simulink model "vehicle_dynamics_system"  (R2012b)
settings: Solver=ode3  StartTime=0.0  StopTime=10.0  FixedStep=T  RelTol=1e-3
PreLoadFcn:
  | init_parameters;
undefined symbols (not defined in the file): CarBody, Differential, Engine, Gearbox, Ground, Suspension, Wheel
libraries: vehicle_dynamics_lib x11, simulink x1
(part 2 of 3)

== matlab function vehicle_dynamics_system/Chassis/Vehicle dynamics ==
  data: q input size=16; q2dot output size=16; stuck output; q1dot input size=16; r_DFL input; FTireFL input; r_DFR input; FTireFR input; r_DRL input; FTireRL input; r_DRR input; FTireRR input; FDamperFL input; FDamperFR input; FDamperRL input; FDamperRR input; gravity input; rFLWheelMountPoint parameter; rFRWheelMountPoint parameter; rRLWheelMountPoint parameter; rRRWheelMountPoint parameter; delta input; rFAirPointOfAttack parameter; rRAirPointOfAttack parameter; FAirDrag input; M_FL input; M_FR input; M_RL input; M_RR input; c_ROLLBARF parameter; c_ROLLBARR parameter; M_BrakeF input; M_BrakeR input; R output; N_Gnd input; m_body parameter; m_wheel parameter; I_body parameter; I_wheel parameter
function [q2dot, stuck, R] ...
    = vehicle_dynamics(q, q1dot, r_DFL, FTireFL, r_DFR, FTireFR, r_DRL, FTireRL, ...
    r_DRR, FTireRR, FDamperFL, FDamperFR, FDamperRL, FDamperRR, gravity, rFLWheelMountPoint, ...
    rFRWheelMountPoint, rRLWheelMountPoint, rRRWheelMountPoint, delta, ...
    rFAirPointOfAttack, rRAirPointOfAttack, FAirDrag, M_FL, M_FR, M_RL, M_RR, ...
    c_ROLLBARF, c_ROLLBARR, M_BrakeF, M_BrakeR, N_Gnd, m_body, m_wheel, I_body, I_wheel)
% This block supports the Embedded MATLAB subset.
% See the help menu for details. 

persistent oldepsFL_zs1dot; if isempty(oldepsFL_zs1dot), oldepsFL_zs1dot = 0; end
persistent oldepsFR_zs1dot; if isempty(oldepsFR_zs1dot), oldepsFR_zs1dot = 0; end
persistent oldepsRL_zs1dot; if isempty(oldepsRL_zs1dot), oldepsRL_zs1dot = 0; end
persistent oldepsRR_zs1dot; if isempty(oldepsRR_zs1dot), oldepsRR_zs1dot = 0; end
persistent stuckFL; if isempty(stuckFL), stuckFL = 0; end
persistent stuckFR; if isempty(stuckFR), stuckFR = 0; end
persistent stuckRL; if isempty(stuckRL), stuckRL = 0; end
persistent stuckRR; if isempty(stuckRR), stuckRR = 0; end

% x_zs = q(1);
% y_zs = q(2);
% z_zs = q(3);
psi_zs = q(4);
theta_zs = q(5);
phi_zs = q(6);
deltaFL_zs = q(7);
deltaFR_zs = q(8);
zFL_zs = q(9);
zFR_zs = q(10);
zRL_zs = q(11);
zRR_zs = q(12);
epsFL_zs = q(13);
epsFR_zs = q(14);
epsRL_zs = q(15);
epsRR_zs = q(16);

% x_zs1dot = q1dot(1);
% y_zs1dot = q1dot(2);
% z_zs1dot = q1dot(3);
psi_zs1dot = q1dot(4);
theta_zs1dot = q1dot(5);
phi_zs1dot = q1dot(6);
deltaFL_zs1dot = q1dot(7);
deltaFR_zs1dot = q1dot(8);
zFL_zs1dot = q1dot(9);
zFR_zs1dot = q1dot(10);
zRL_zs1dot = q1dot(11);
zRR_zs1dot = q1dot(12);
epsFL_zs1dot = q1dot(13);
epsFR_zs1dot = q1dot(14);
epsRL_zs1dot = q1dot(15);
epsRR_zs1dot = q1dot(16);

xTireFL = FTireFL(1);
yTireFL = FTireFL(2);
zTireFL = FTireFL(3);

xTireFR = FTireFR(1);
yTireFR = FTireFR(2);
zTireFR = FTireFR(3);

xTireRL = FTireRL(1);
yTireRL = FTireRL(2);
zTireRL = FTireRL(3);

xTireRR = FTireRR(1);
yTireRR = FTireRR(2);
zTireRR = FTireRR(3);

%Calculate anti roll bar forces
dsuspF = zFL_zs - zFR_zs;
dsuspR = zRL_zs - zRR_zs;

F_RBF = dsuspF*c_ROLLBARF;
F_RBR = dsuspR*c_ROLLBARR;

%Calculate chassis rotation matrix
R=zeros(3,3);

t1 = cos(psi_zs);
t2 = cos(theta_zs);
t4 = sin(psi_zs);
t5 = cos(phi_zs);
t7 = sin(theta_zs);
t8 = t1 * t7;
t9 = sin(phi_zs);
t17 = t7 * t4;
R(1,1) = t1 * t2;
R(1,2) = -t4 * t5 + t8 * t9;
R(1,3) = t4 * t9 + t8 * t5;
R(2,1) = t2 * t4;
R(2,2) = t1 * t5 + t17 * t9;
R(2,3) = -t1 * t9 + t17 * t5;
R(3,1) = -t7;
R(3,2) = t2 * t9;
R(3,3) = t2 * t5;

cd = cos(deltaFL_zs);
sd = sin(deltaFL_zs);
%Calculate front wheel rotation matrix
Rf = R*[cd, -sd, 0;
        sd, cd, 0;
        0, 0, 1];

%Calculate necessary braking torque
r_fwdF = Rf(:,1);
r_fwdR = R(:,1);

if( M_BrakeF > 0 || M_BrakeR > 0 )
    
    whltrqFL = -FTireFL.'*r_fwdF*r_DFL+M_FL;
	whltrqFR = -FTireFR.'*r_fwdF*r_DFR+M_FR;
	whltrqRL = -FTireRL.'*r_fwdR*r_DRL+M_RL;
	whltrqRR = -FTireRR.'*r_fwdR*r_DRR+M_RR;
    
	M_FL = M_FL - sign(epsFL_zs1dot)*M_BrakeF;
    M_FR = M_FR - sign(epsFR_zs1dot)*M_BrakeF;
    M_RL = M_RL - sign(epsRL_zs1dot)*M_BrakeR;
    M_RR = M_RR - sign(epsRR_zs1dot)*M_BrakeR;
    
    %FL
    if( abs(whltrqFL) < M_BrakeF )
        if( sign(oldepsFL_zs1dot) ~= sign(epsFL_zs1dot) )
            stuckFL = 1;
        end
    else
        stuckFL = 0;
    end
    
    %FR
    if( abs(whltrqFR) < M_BrakeF )
        if( sign(oldepsFR_zs1dot) ~= sign(epsFR_zs1dot) )
            stuckFR = 1;
        end
    else
        stuckFR = 0;
    end
    
    %RL
    if( abs(whltrqRL) < M_BrakeR )
        if( sign(oldepsRL_zs1dot) ~= sign(epsRL_zs1dot) )
            stuckRL = 1;
        end
    else
        stuckRL = 0;
    end
    
    %RR
    if( abs(whltrqRR) < M_BrakeR )
        if( sign(oldepsRR_zs1dot) ~= sign(epsRR_zs1dot) )
            stuckRR = 1;
        end
    else
        stuckRR = 0;
    end
else
    stuckFL = 0;
    stuckFR = 0;
    stuckRL = 0;
    stuckRR = 0;
end
    
g = gravity;

n_gndFL_X = N_Gnd(1);
n_gndFL_Y = N_Gnd(2);
n_gndFL_Z = N_Gnd(3);

n_gndFR_X = N_Gnd(4);
n_gndFR_Y = N_Gnd(5);
n_gndFR_Z = N_Gnd(6);

n_gndRL_X = N_Gnd(7);
n_gndRL_Y = N_Gnd(8);
n_gndRL_Z = N_Gnd(9);

n_gndRR_X = N_Gnd(10);
n_gndRR_Y = N_Gnd(11);
n_gndRR_Z = N_Gnd(12);

F_DSFL = FDamperFL + F_RBF;
F_DSFR = FDamperFR - F_RBF;
F_DSRL = FDamperRL + F_RBR;
F_DSRR = FDamperRR - F_RBF;

F_AIRFRONT_X = FAirDrag(1);
F_AIRFRONT_Z = FAirDrag(2);

F_AIRREAR_X = FAirDrag(3);
F_AIRREAR_Z = FAirDrag(4);

r_wheelMntFL_X = rFLWheelMountPoint(1);
r_wheelMntFL_Y = rFLWheelMountPoint(2);
r_wheelMntFL_Z = rFLWheelMountPoint(3);

r_wheelMntFR_X = rFRWheelMountPoint(1);
r_wheelMntFR_Y = rFRWheelMountPoint(2);
r_wheelMntFR_Z = rFRWheelMountPoint(3);

r_wheelMntRL_X = rRLWheelMountPoint(1);
r_wheelMntRL_Y = rRLWheelMountPoint(2);
r_wheelMntRL_Z = rRLWheelMountPoint(3);

r_wheelMntRR_X = rRRWheelMountPoint(1);
r_wheelMntRR_Y = rRRWheelMountPoint(2);
r_wheelMntRR_Z = rRRWheelMountPoint(3);

r_airFront_X = rFAirPointOfAttack(1);
r_airFront_Y = rFAirPointOfAttack(2);
r_airFront_Z = rFAirPointOfAttack(3);

r_airRear_X = rRAirPointOfAttack(1);
r_airRear_Y = rRAirPointOfAttack(2);
r_airRear_Z = rRAirPointOfAttack(3);

I_body_xx = I_body(1,1);
I_body_yy = I_body(2,2);
I_body_zz = I_body(3,3);

I_wheel_xx = I_wheel(1,1);
I_wheel_yy = I_wheel(2,2);
I_wheel_zz = I_wheel(3,3);

deltaFR = delta;
deltaFL = delta;

gg = zeros(14,15);

%Warning: the function names {F_AIRFRONT_Z, F_AIRREAR_Z, M_FL, F_DSFR, F_DSRL, F_DSRR, F_AIRFRONT_X, M_FR, F_DSFL, F_AIRREAR_X, xTireFL, yTireFL, zTireFL, M_RL, M_RR, xTireFR, yTireFR, zTireFR, xTireRL, yTireRL, zTireRL, xTireRR, yTireRR, zTireRR} are not recognized in the target language
t2 = m_body + 4 * m_wheel;
t3 = m_wheel * r_wheelMntRL_Z;
t4 = sin(psi_zs);
t5 = sin(theta_zs);
t6 = t4 * t5;
t7 = cos(phi_zs);
t8 = t6 * t7;
t10 = m_wheel * zRL_zs;
t12 = cos(psi_zs);
t13 = sin(phi_zs);
t14 = t12 * t13;
t16 = m_wheel * zFR_zs;
t18 = m_wheel * r_wheelMntFL_Y;
t19 = t12 * t7;
t21 = m_wheel * t4;
t22 = cos(theta_zs);
t23 = t22 * r_wheelMntRR_X;
t25 = m_wheel * r_wheelMntRR_Y;
t27 = t22 * r_wheelMntFL_X;
t29 = m_wheel * zFL_zs;
t31 = m_wheel * r_wheelMntFR_Y;
t32 = t6 * t13;
t34 = m_wheel * r_wheelMntFR_Z;
t36 = t22 * r_wheelMntFR_X;
t39 = m_wheel * zRR_zs;
t41 = -t3 * t8 - t10 * t8 + t3 * t14 + t16 * t14 - t18 * t19 - t21 * t23 - t25 * t19 - t21 * t27 + t29 * t14 - t31 * t32 + t34 * t14 - t21 * t36 - t31 * t19 + t39 * t14;
t43 = t22 * r_wheelMntRL_X;
t45 = m_wheel * r_wheelMntRL_Y;
t49 = m_wheel * r_wheelMntFL_Z;
t51 = m_wheel * r_wheelMntRR_Z;
t60 = t10 * t14 - t21 * t43 - t45 * t19 - t16 * t8 - t34 * t8 - t49 * t8 + t51 * t14 - t18 * t32 - t45 * t32 - t29 * t8 + t49 * t14 - t51 * t8 - t25 * t32 - t39 * t8;
t61 = t41 + t60;
t62 = t12 * t22;
t63 = t62 * t7;
t65 = t62 * t13;
t68 = m_wheel * t12;
t69 = t5 * r_wheelMntFR_X;
t76 = t5 * r_wheelMntRL_X;
t80 = t5 * r_wheelMntFL_X;
t83 = t5 * r_wheelMntRR_X;
t86 = t16 * t63 + t25 * t65 + t34 * t63 - t68 * t69 + t31 * t65 + t39 * t63 + t3 * t63 + t10 * t63 + t45 * t65 - t68 * t76 + t29 * t63 + t18 * t65 - t68 * t80 + t49 * t63 - t68 * t83 + t51 * t63;
t87 = t4 * t7;
t90 = t4 * t13;
t92 = t12 * t5;
t93 = t92 * t13;
t96 = t92 * t7;
t104 = t29 * t87 + t49 * t87 + t31 * t90 - t16 * t93 - t34 * t93 + t25 * t96 + t16 * t87 + t31 * t96 - t39 * t93 + t39 * t87 + t45 * t96 - t3 * t93;
t117 = -t10 * t93 + t3 * t87 + t10 * t87 + t18 * t96 + t45 * t90 + t34 * t87 - t29 * t93 + t18 * t90 - t49 * t93 + t25 * t90 + t51 * t87 - t51 * t93;
t118 = t104 + t117;
t119 = t5 * t7;
t122 = t68 * t119 + t21 * t13;
t123 = m_wheel * zFR_zs1dot;
t124 = t87 * phi_zs1dot;
t127 = t31 * t12;
t128 = psi_zs1dot ^ 2;
t129 = t128 * t5;
t130 = t129 * t13;
t132 = t31 * t4;
t133 = psi_zs1dot * t22;
t134 = theta_zs1dot * t13;
t135 = t133 * t134;
t138 = t25 * t12;
t139 = psi_zs1dot * t13;
t140 = t139 * phi_zs1dot;
t143 = t4 * t128;
t144 = t143 * t7;
t146 = t143 * t13;
t148 = phi_zs1dot ^ 2;
t149 = t90 * t148;
t151 = t39 * t12;
t152 = psi_zs1dot * t7;
t153 = t152 * phi_zs1dot;
t156 = t18 * t12;
t159 = m_wheel * zFL_zs1dot;
t161 = t12 * psi_zs1dot * t13;
t164 = theta_zs1dot ^ 2;
t165 = t22 * t164;
t166 = t165 * r_wheelMntRR_X;
t168 = t49 * t4;
t169 = theta_zs1dot * t7;
t170 = t133 * t169;
t173 = psi_zs1dot * t5;
t174 = t13 * phi_zs1dot;
t175 = t173 * t174;
t178 = t49 * t12;
t181 = t5 * t13;
t182 = t181 * t148;
t184 = t25 * t4;
t187 = t7 * phi_zs1dot;
t188 = t173 * t187;
t191 = t128 * t22;
t192 = t191 * r_wheelMntFL_X;
t194 = 0.2e1 * t123 * t124 - t127 * t130 - 0.2e1 * t132 * t135 + 0.2e1 * t138 * t140 + t31 * t144 - t39 * t146 - t39 * t149 + 0.2e1 * t151 * t153 + 0.2e1 * t156 * t140 + 0.2e1 * t159 * t161 - t68 * t166 - 0.2e1 * t168 * t170 + 0.2e1 * t168 * t175 + 0.2e1 * t178 * t153 - t156 * t182 - 0.2e1 * t184 * t135 - 0.2e1 * t184 * t188 - t68 * t192;
t198 = t34 * t12;
t199 = t119 * t148;
t202 = t191 * r_wheelMntFR_X;
t204 = t45 * t12;
t206 = t45 * t4;
t211 = m_wheel * zRL_zs1dot;
t212 = t211 * t12;
t213 = t181 * phi_zs1dot;
t218 = t16 * t12;
t219 = t129 * t7;
t221 = t165 * r_wheelMntFR_X;
t225 = t5 * t164;
t226 = t225 * t13;
t228 = t22 * theta_zs1dot;
t229 = t228 * t187;
t232 = t225 * t7;
t237 = 0.2e1 * t127 * t140 - t34 * t146 - t198 * t199 - t16 * t146 - t68 * t202 - t204 * t130 - 0.2e1 * t206 * t135 - 0.2e1 * t206 * t188 - 0.2e1 * t212 * t213 - t49 * t149 - t49 * t146 - t218 * t219 - t68 * t221 - 0.2e1 * t132 * t188 - t127 * t226 + 0.2e1 * t127 * t229 - t151 * t232 - t127 * t182 + 0.2e1 * t198 * t153;
t240 = t29 * t4;
t246 = xTireFL;
t247 = t34 * t4;
t253 = t18 * t4;
t261 = m_wheel * zRR_zs1dot;
t262 = t261 * t4;
t263 = t173 * t7;
t266 = t261 * t12;
t267 = t228 * t7;
t272 = t51 * t12;
t273 = t228 * t174;
t282 = -t198 * t219 - 0.2e1 * t240 * t170 + 0.2e1 * t240 * t175 - t204 * t226 - t246 - 0.2e1 * t247 * t170 + 0.2e1 * t247 * t175 - t178 * t199 - 0.2e1 * t253 * t135 - 0.2e1 * t253 * t188 - t156 * t226 + 0.2e1 * t218 * t153 - 0.2e1 * t262 * t263 + 0.2e1 * t266 * t267 - 0.2e1 * t266 * t213 - 0.2e1 * t272 * t273 - 0.2e1 * t151 * t273 + 0.2e1 * t156 * t229 + 0.2e1 * t211 * t161;
t285 = t191 * r_wheelMntRL_X;
t288 = t10 * t12;
t292 = t21 * psi_zs1dot;
t293 = t5 * theta_zs1dot;
t294 = t293 * r_wheelMntRL_X;
t297 = t3 * t12;
t299 = t87 * t148;
t302 = t123 * t4;
t305 = t123 * t12;
t312 = t16 * t4;
t316 = t3 * t4;
t321 = t29 * t12;
t323 = 0.2e1 * t211 * t124 - t68 * t285 - t138 * t130 - 0.2e1 * t288 * t273 - t288 * t199 + 0.2e1 * t292 * t294 - t297 * t219 + t18 * t299 - t178 * t219 - 0.2e1 * t302 * t263 + 0.2e1 * t305 * t267 - 0.2e1 * t305 * t213 + t31 * t299 - t151 * t219 - 0.2e1 * t312 * t170 - t272 * t199 - 0.2e1 * t316 * t170 + 0.2e1 * t316 * t175 - t321 * t199;
t329 = t293 * r_wheelMntFL_X;
t332 = t39 * t4;
t338 = t51 * t4;
t341 = F_AIRFRONT_Z;
t342 = t341 * t12;
t345 = t10 * t4;
t351 = t191 * r_wheelMntRR_X;
t360 = -t178 * t232 - 0.2e1 * t178 * t273 + 0.2e1 * t292 * t329 - 0.2e1 * t332 * t170 + 0.2e1 * t332 * t175 - t272 * t219 - 0.2e1 * t338 * t170 - t342 * t119 - t288 * t219 - 0.2e1 * t345 * t170 + 0.2e1 * t345 * t175 + t25 * t144 - t68 * t351 + t25 * t299 - t51 * t146 + 0.2e1 * t338 * t175 + 0.2e1 * t261 * t124 + t45 * t144;
t361 = t165 * r_wheelMntRL_X;
t379 = t293 * r_wheelMntFR_X;
t387 = xTireRL;
t388 = xTireFR;
t389 = F_AIRREAR_Z;
t390 = t389 * t4;
t392 = -t68 * t361 - t3 * t146 - t321 * t232 - 0.2e1 * t321 * t273 + 0.2e1 * t321 * t153 + 0.2e1 * t159 * t124 - t51 * t149 + 0.2e1 * t261 * t161 - t272 * t232 - t297 * t232 - 0.2e1 * t297 * t273 - t218 * t199 + 0.2e1 * t292 * t379 + 0.2e1 * t204 * t229 - t204 * t182 + 0.2e1 * t297 * t153 - t387 - t388 - t390 * t13;
t394 = F_AIRREAR_X;
t401 = t159 * t4;
t404 = t159 * t12;
t414 = t165 * r_wheelMntFL_X;
t425 = t389 * t12;
t427 = -t62 * t394 + 0.2e1 * t204 * t140 + 0.2e1 * t288 * t153 - t3 * t149 - 0.2e1 * t401 * t263 + 0.2e1 * t404 * t267 - 0.2e1 * t404 * t213 - t321 * t219 - t29 * t149 - t198 * t232 - 0.2e1 * t198 * t273 - t68 * t414 + t18 * t144 + 0.2e1 * t312 * t175 - t218 * t232 - 0.2e1 * t218 * t273 - t34 * t149 + 0.2e1 * t123 * t161 - t425 * t119;
t439 = t211 * t4;
t445 = t293 * r_wheelMntRR_X;
t450 = xTireRR;
t452 = t341 * t4;
t454 = F_AIRFRONT_X;
t456 = -t138 * t226 - t297 * t199 - t288 * t232 - t156 * t130 - t29 * t146 - t10 * t146 - t10 * t149 + 0.2e1 * t272 * t153 - t16 * t149 + t45 * t299 - 0.2e1 * t439 * t263 + 0.2e1 * t212 * t267 - t151 * t199 + 0.2e1 * t292 * t445 + 0.2e1 * t138 * t229 - t450 - t138 * t182 - t452 * t13 - t62 * t454;
t474 = t16 * t96 + t31 * t93 + t25 * t93 + t51 * t96 + t18 * t93 + t49 * t96 + t29 * t96 + t10 * t96 + t45 * t93 + t3 * t96 + t34 * t96 - t45 * t87 + t68 * t27 - t18 * t87;
t489 = t68 * t36 - t31 * t87 + t34 * t90 + t16 * t90 + t68 * t23 - t25 * t87 + t51 * t90 + t39 * t90 + t29 * t90 + t68 * t43 + t10 * t90 + t3 * t90 + t39 * t96 + t49 * t90;
t490 = t474 + t489;
t493 = t4 * t22;
t494 = t493 * t7;
t496 = t493 * t13;
t510 = -t21 * t80 - t21 * t69 + t16 * t494 + t25 * t496 - t21 * t83 - t21 * t76 + t18 * t496 + t49 * t494 + t3 * t494 + t10 * t494 + t45 * t496 + t31 * t496 + t34 * t494 + t39 * t494 + t51 * t494 + t29 * t494;
t523 = -t29 * t19 - t18 * t14 - t31 * t14 - t34 * t19 - t16 * t19 - t34 * t32 - t16 * t32 + t25 * t8 - t25 * t14 - t51 * t19 - t39 * t19 + t18 * t8;
t536 = -t49 * t32 - t3 * t32 + t45 * t8 - t3 * t19 - t10 * t19 + t31 * t8 - t45 * t14 - t51 * t32 - t39 * t32 - t29 * t32 - t49 * t19 - t10 * t32;
t537 = t523 + t536;
t540 = t21 * t119 - t68 * t13;
t547 = t14 * t148;
t549 = t12 * t128;
t550 = t549 * t13;
t565 = yTireFL;
t567 = -0.2e1 * t272 * t175 - t338 * t232 - 0.2e1 * t338 * t273 - t338 * t199 + t10 * t547 + t10 * t550 - t316 * t219 + 0.2e1 * t266 * t263 + 0.2e1 * t262 * t267 - t206 * t226 - t206 * t130 + 0.2e1 * t204 * t135 + t51 * t550 + t51 * t547 + t39 * t547 - t184 * t130 - t565 - t132 * t130;
t576 = t68 * psi_zs1dot;
t581 = t549 * t7;
t583 = t19 * t148;
t598 = t34 * t550 + t34 * t547 + 0.2e1 * t312 * t153 - t168 * t232 - 0.2e1 * t168 * t273 - t21 * t221 - 0.2e1 * t576 * t329 - 0.2e1 * t321 * t175 - t18 * t581 - t18 * t583 + t49 * t550 - t184 * t182 - t21 * t166 - t25 * t581 + 0.2e1 * t198 * t170 - 0.2e1 * t198 * t175 - t247 * t232 - 0.2e1 * t247 * t273 + 0.2e1 * t439 * t267;
t609 = t4 * psi_zs1dot * t13;
t612 = t19 * phi_zs1dot;
t637 = -0.2e1 * t439 * t213 - t316 * t232 - 0.2e1 * t262 * t213 - t332 * t219 - 0.2e1 * t178 * t175 + 0.2e1 * t159 * t609 - 0.2e1 * t159 * t612 + 0.2e1 * t151 * t170 - 0.2e1 * t151 * t175 - 0.2e1 * t302 * t213 - t312 * t219 + 0.2e1 * t218 * t170 - 0.2e1 * t218 * t175 + 0.2e1 * t316 * t153 + 0.2e1 * t261 * t609 + t3 * t550 + 0.2e1 * t138 * t135 + 0.2e1 * t138 * t188 + 0.2e1 * t184 * t229;
t644 = yTireRR;
t664 = -t184 * t226 - 0.2e1 * t401 * t213 - t240 * t219 - t31 * t581 - t31 * t583 - t644 + 0.2e1 * t297 * t170 - 0.2e1 * t261 * t612 + t39 * t550 - t345 * t199 + t49 * t547 - t253 * t130 - t132 * t226 - t132 * t182 + 0.2e1 * t247 * t153 - t247 * t219 + 0.2e1 * t272 * t170 + 0.2e1 * t211 * t609 + 0.2e1 * t253 * t140;
t669 = yTireRL;
t697 = 0.2e1 * t404 * t263 - t669 + 0.2e1 * t401 * t267 + 0.2e1 * t156 * t135 - t312 * t232 - t312 * t199 - 0.2e1 * t576 * t379 - 0.2e1 * t211 * t612 - 0.2e1 * t332 * t273 - t332 * t232 - t332 * t199 - 0.2e1 * t576 * t445 + 0.2e1 * t184 * t140 + 0.2e1 * t332 * t153 - t390 * t119 + 0.2e1 * t204 * t188 + 0.2e1 * t127 * t135 + 0.2e1 * t127 * t188;
t723 = -t452 * t119 - 0.2e1 * t288 * t175 - t345 * t232 - 0.2e1 * t345 * t273 + t29 * t550 + t29 * t547 - t21 * t192 - t21 * t285 - t253 * t226 + 0.2e1 * t253 * t229 - t253 * t182 + 0.2e1 * t321 * t170 - t240 * t232 - t21 * t414 - t21 * t361 - t45 * t581 - t21 * t351 + 0.2e1 * t338 * t153 + 0.2e1 * t240 * t153;
t741 = yTireFR;
t754 = t16 * t550 + 0.2e1 * t123 * t609 - 0.2e1 * t123 * t612 - t21 * t202 - t316 * t199 - t345 * t219 + 0.2e1 * t288 * t170 - t493 * t454 + t425 * t13 + 0.2e1 * t212 * t263 - 0.2e1 * t316 * t273 - t741 + 0.2e1 * t178 * t170 - t45 * t583 - 0.2e1 * t576 * t294 + 0.2e1 * t206 * t140 + 0.2e1 * t132 * t140 - t247 * t199 - 0.2e1 * t312 * t273;
t783 = -t25 * t583 + 0.2e1 * t156 * t188 - t168 * t199 - 0.2e1 * t240 * t273 - t240 * t199 + 0.2e1 * t132 * t229 + 0.2e1 * t345 * t153 - 0.2e1 * t297 * t175 - t338 * t219 + 0.2e1 * t206 * t229 - t206 * t182 + t3 * t547 + 0.2e1 * t168 * t153 - t168 * t219 + t16 * t547 + 0.2e1 * t305 * t263 + 0.2e1 * t302 * t267 - t493 * t394 + t342 * t13;
t787 = m_wheel * t5;
t788 = t7 * r_wheelMntFL_Z;
t790 = t7 * zFL_zs;
t792 = m_wheel * t22;
t794 = t792 * r_wheelMntFL_X;
t795 = t7 * r_wheelMntRL_Z;
t797 = t13 * r_wheelMntFR_Y;
t799 = t7 * r_wheelMntFR_Z;
t801 = t7 * r_wheelMntRR_Z;
t803 = t7 * zRR_zs;
t805 = t7 * zFR_zs;
t807 = t13 * r_wheelMntRR_Y;
t809 = t7 * zRL_zs;
t811 = t13 * r_wheelMntRL_Y;
t813 = t13 * r_wheelMntFL_Y;
t815 = t792 * r_wheelMntRL_X;
t816 = t792 * r_wheelMntFR_X;
t817 = -t787 * t788 - t787 * t790 - t792 * r_wheelMntRR_X - t794 - t787 * t795 - t787 * t797 - t787 * t799 - t787 * t801 - t787 * t803 - t787 * t805 - t787 * t807 - t787 * t809 - t787 * t811 - t787 * t813 - t815 - t816;
t818 = t13 * r_wheelMntFL_Z;
t820 = t13 * zRR_zs;
t822 = t13 * r_wheelMntRL_Z;
t824 = t13 * zFR_zs;
t826 = t7 * r_wheelMntFR_Y;
t828 = t13 * r_wheelMntRR_Z;
t830 = t13 * r_wheelMntFR_Z;
t832 = t7 * r_wheelMntRR_Y;
t834 = t13 * zRL_zs;
t836 = t7 * r_wheelMntRL_Y;
t838 = t13 * zFL_zs;
t840 = t7 * r_wheelMntFL_Y;
t842 = -t792 * t818 - t792 * t820 - t792 * t822 - t792 * t824 + t792 * t826 - t792 * t828 - t792 * t830 + t792 * t832 - t792 * t834 + t792 * t836 - t792 * t838 + t792 * t840;
t843 = t792 * t7;
t847 = t164 * t13;
t850 = t787 * theta_zs1dot;
t854 = t164 * t7;
t867 = t7 * t148;
t870 = zTireFL;
t871 = t13 * t148;
t881 = -0.2e1 * t787 * t169 * zFL_zs1dot - t792 * t847 * r_wheelMntFL_Y - 0.2e1 * t850 * t187 * r_wheelMntFL_Y - t792 * t854 * r_wheelMntFL_Z - t792 * t847 * r_wheelMntRR_Y - 0.2e1 * t850 * t187 * r_wheelMntRR_Y - t792 * t854 * r_wheelMntRR_Z + 0.2e1 * t850 * t174 * r_wheelMntRL_Z - t792 * t867 * zFR_zs - t870 - t792 * t871 * r_wheelMntRL_Y - t792 * t854 * zRL_zs + 0.2e1 * t850 * t174 * zRL_zs - t792 * t867 * zRL_zs;
t905 = m_wheel * g;
t915 = -0.2e1 * t850 * t187 * r_wheelMntRL_Y - t792 * t854 * r_wheelMntRL_Z - 0.2e1 * t792 * t174 * zFR_zs1dot - t792 * t871 * r_wheelMntFR_Y - t792 * t847 * r_wheelMntRL_Y - 0.2e1 * t787 * t169 * zFR_zs1dot + t5 * t454 - t792 * t854 * zFR_zs - t792 * t871 * r_wheelMntRR_Y - 0.2e1 * t787 * t169 * zRR_zs1dot + (4 * t905) + 0.2e1 * t850 * t174 * r_wheelMntFL_Z - t792 * t867 * r_wheelMntFL_Z - t792 * t867 * zRR_zs + t5 * t394;
t918 = t22 * t7;
t929 = zTireFR;
t946 = (m_body * g) - t918 * t389 - t792 * t854 * r_wheelMntFR_Z + 0.2e1 * t850 * t174 * r_wheelMntFR_Z - t792 * t867 * r_wheelMntFR_Z - t792 * t854 * zFL_zs - t929 + 0.2e1 * t850 * t174 * zFL_zs - 0.2e1 * t792 * t174 * zFL_zs1dot + t787 * t164 * r_wheelMntFL_X + t787 * t164 * r_wheelMntRR_X + t787 * t164 * r_wheelMntRL_X + t787 * t164 * r_wheelMntFR_X - t792 * t867 * zFL_zs;
t964 = zTireRR;
t965 = zTireRL;
t981 = 0.2e1 * t850 * t174 * r_wheelMntRR_Z - t792 * t867 * r_wheelMntRR_Z - t792 * t854 * zRR_zs + 0.2e1 * t850 * t174 * zFR_zs - t792 * t847 * r_wheelMntFR_Y - 0.2e1 * t850 * t187 * r_wheelMntFR_Y - t792 * t871 * r_wheelMntFL_Y - t964 - t965 + 0.2e1 * t850 * t174 * zRR_zs - 0.2e1 * t792 * t174 * zRR_zs1dot - t792 * t867 * r_wheelMntRL_Z - 0.2e1 * t787 * t169 * zRL_zs1dot - 0.2e1 * t792 * t174 * zRL_zs1dot - t918 * t341;
t984 = cos(epsFL_zs);
t985 = I_wheel_zz * t984;
t986 = t985 * t22;
t987 = cos(deltaFL);
t988 = sin(epsFL_zs);
t989 = t987 * t988;
t990 = t989 * t119;
t993 = t22 ^ 2;
t994 = I_wheel_xx * t993;
t995 = cos(deltaFR);
t996 = t995 ^ 2;
t997 = cos(epsFR_zs);
t998 = t997 ^ 2;
t999 = t996 * t998;
t1002 = t987 ^ 2;
t1003 = I_wheel_zz * t1002;
t1004 = t7 ^ 2;
t1005 = t993 * t1004;
t1007 = zFL_zs ^ 2;
t1008 = m_wheel * t1007;
t1010 = r_wheelMntFL_Z ^ 2;
t1011 = m_wheel * t1010;
t1013 = t984 ^ 2;
t1014 = I_wheel_zz * t1013;
t1015 = t1002 * t993;
t1018 = I_wheel_xx * t998;
t1021 = r_wheelMntRR_Y ^ 2;
t1022 = m_wheel * t1021;
t1024 = I_wheel_zz * t1004;
t1025 = t998 * t993;
t1028 = I_wheel_xx * t1004;
t1029 = cos(epsRR_zs);
t1030 = t1029 ^ 2;
t1031 = t993 * t1030;
t1033 = r_wheelMntRL_Y ^ 2;
t1034 = m_wheel * t1033;
t1036 = I_wheel_xx * t997;
t1037 = sin(deltaFR);
t1038 = t1036 * t1037;
t1039 = sin(epsFR_zs);
t1040 = t13 * t1039;
t1041 = t7 * t993;
t1042 = t1040 * t1041;
t1045 = cos(epsRL_zs);
t1046 = t1045 ^ 2;
t1047 = I_wheel_xx * t1046;
t1048 = zRL_zs ^ 2;
t1049 = m_wheel * t1048;
t1050 = r_wheelMntFR_Y ^ 2;
t1051 = m_wheel * t1050;
t1052 = -0.2e1 * t986 * t990 - 0.2e1 * t994 * t999 + t1003 * t1005 - t1008 * t1005 - t1011 * t1005 + 0.2e1 * t1014 * t1015 - 0.2e1 * t1018 * t1005 + t1022 * t1005 + 0.2e1 * t1024 * t1025 - t1028 * t1031 + t1034 * t1005 + 0.2e1 * t1038 * t1042 + t1047 + t1049 + t1051 + t1022;
t1053 = I_wheel_yy * t1002;
t1054 = I_wheel_zz * t1030;
t1055 = I_wheel_xx * t1030;
t1056 = r_wheelMntRR_Z ^ 2;
t1057 = m_wheel * t1056;
t1058 = r_wheelMntFL_Y ^ 2;
t1059 = m_wheel * t1058;
t1060 = I_wheel_zz * t996;
t1063 = 2 * t49 * zFL_zs;
t1064 = I_wheel_zz * t993;
t1067 = t49 * t13;
t1071 = t996 * t993;
t1072 = t1071 * t1004;
t1074 = I_wheel_zz * t998;
t1075 = t1074 * t22;
t1076 = t995 * t1037;
t1080 = I_wheel_zz * t1046;
t1081 = t1036 * t22;
t1082 = t995 * t1039;
t1083 = t1082 * t119;
t1086 = t45 * t7;
t1090 = I_body_xx - t1053 - t1054 + t1055 + t1057 + t1059 + t1060 - t1014 * t993 + t1063 - 0.2e1 * t1064 * t1004 + t1011 - 0.2e1 * t1067 * t840 * t993 + t1018 * t1072 - 0.2e1 * t1075 * t1076 * t181 - t1080 + 0.2e1 * t1081 * t1083 - 0.2e1 * t1086 * t834 * t993;
t1092 = I_wheel_xx * t1013;
t1093 = t1015 * t1004;
t1096 = r_wheelMntFL_Y * t5 * t13;
t1099 = zFR_zs ^ 2;
t1100 = m_wheel * t1099;
t1101 = 0.2e1 * I_wheel_yy;
t1102 = zRR_zs ^ 2;
t1103 = m_wheel * t1102;
t1104 = t1004 * zRL_zs;
t1108 = r_wheelMntRL_Z ^ 2;
t1109 = m_wheel * t1108;
t1112 = r_wheelMntFR_Y * t5 * t13;
t1116 = t918 * r_wheelMntRR_X;
t1119 = t1014 * t1002;
t1120 = I_wheel_xx * t984;
t1121 = sin(deltaFL);
t1122 = t1120 * t1121;
t1123 = t7 * t988;
t1124 = t13 * t993;
t1125 = t1123 * t1124;
t1128 = t45 * t13;
t1132 = t1004 * r_wheelMntFR_Z;
t1133 = t1132 * t993;
t1137 = t1092 * t1093 + 0.2e1 * t794 * t1096 + t1100 + t1003 + t1101 + t1103 - 0.2e1 * t3 * t1104 * t993 + t1109 + t1008 - I_body_xx * t993 + 0.2e1 * t816 * t1112 + 0.2e1 * t51 * t5 * t1116 - t1119 + 0.2e1 * t1122 * t1125 - 0.2e1 * t1128 * t795 * t993 - 0.2e1 * t16 * t1133 - t1014 * t1093;
t1138 = m_wheel * t993;
t1139 = r_wheelMntFL_X ^ 2;
t1143 = 2 * t51 * zRR_zs;
t1144 = t1014 * t22;
t1145 = t987 * t1121;
t1146 = t1145 * t181;
t1149 = t16 * t7;
t1153 = t25 * t5;
t1154 = t13 * t22;
t1155 = t1154 * r_wheelMntRR_X;
t1158 = r_wheelMntFR_Z * t5;
t1159 = t1158 * t7;
t1162 = I_body_yy * t993;
t1163 = 0.2e1 * I_wheel_zz;
t1164 = zFL_zs * t5;
t1165 = t1164 * t7;
t1168 = I_wheel_zz * t997;
t1169 = t1168 * t1037;
t1172 = t1092 * t1002;
t1177 = t1138 * t1139 + t1018 * t993 + t1143 - 0.2e1 * t1144 * t1146 - 0.2e1 * t1149 * t797 * t993 + 0.2e1 * t1153 * t1155 + 0.2e1 * t816 * t1159 + t1162 + t1034 + t1163 + 0.2e1 * t794 * t1165 - 0.2e1 * t1169 * t1042 + t1172 + t1080 * t1005 + t1051 * t1005 - t1047 * t1005 - t1103 * t1005;
t1184 = I_wheel_yy * t996;
t1186 = r_wheelMntFR_Z ^ 2;
t1187 = m_wheel * t1186;
t1201 = zRL_zs * t5;
t1202 = t1201 * t7;
t1205 = t1092 * t22;
t1208 = -t1100 * t1005 - t1049 * t1005 + 0.2e1 * t1014 * t1005 - t1184 * t1005 - t1187 * t1005 - t1057 * t1005 - t1053 * t1005 - 0.2e1 * t1092 * t1005 + 0.2e1 * t1074 * t1071 - 0.2e1 * t1092 * t1015 + t1059 * t1005 - t1109 * t1005 + t1060 * t1005 + t1054 * t1005 + 0.2e1 * t815 * t1202 + 0.2e1 * t1205 * t1146;
t1209 = t39 * t13;
t1210 = t832 * t993;
t1213 = zRR_zs * t1004;
t1214 = t1213 * t993;
t1217 = I_wheel_xx * t22;
t1219 = t1037 * t5;
t1220 = t13 * t998;
t1224 = t1217 * t1045;
t1225 = sin(epsRL_zs);
t1226 = t1225 * t5;
t1227 = t1226 * t7;
t1230 = t1168 * t22;
t1233 = r_wheelMntFL_Z * t5;
t1234 = t1233 * t7;
t1245 = I_wheel_yy * t993;
t1250 = 2 * t34 * zFR_zs;
t1251 = -t1184 - 0.2e1 * t1209 * t1210 - 0.2e1 * t51 * t1214 + 0.2e1 * t1217 * t995 * t1219 * t1220 + 0.2e1 * t1224 * t1227 - 0.2e1 * t1230 * t1083 + 0.2e1 * t794 * t1234 + t1187 + t1092 * t993 - t1074 * t993 + 0.2e1 * t1184 * t993 - 0.2e1 * t1064 * t996 + t1064 * t1030 - t1022 * t993 + 0.2e1 * t1245 * t1002 - t1162 * t1004 + t1250;
t1253 = t1018 * t996;
t1258 = I_wheel_zz * t22;
t1259 = t1258 * t1121;
t1260 = t987 * t5;
t1264 = r_wheelMntFR_X ^ 2;
t1266 = zFL_zs * t1004;
t1267 = t1266 * t993;
t1270 = t39 * t5;
t1273 = t18 * t13;
t1277 = t16 * t5;
t1278 = t918 * r_wheelMntFR_X;
t1281 = t1258 * t995;
t1282 = t1219 * t13;
t1289 = t1258 * t1045;
t1292 = t45 * t5;
t1293 = t1154 * r_wheelMntRL_X;
t1296 = t1120 * t22;
t1299 = t1253 - t994 * t1030 + 0.4e1 * t1028 * t993 - t1074 * t1072 + 0.2e1 * t1259 * t1260 * t13 + t1138 * t1264 - 0.2e1 * t49 * t1267 + 0.2e1 * t1270 * t1116 - 0.2e1 * t1273 * t790 * t993 + 0.2e1 * t1277 * t1278 + 0.2e1 * t1281 * t1282 + t1064 * t1046 - t1051 * t993 - 0.2e1 * t1245 * t1004 - 0.2e1 * t1289 * t1227 + 0.2e1 * t1292 * t1293 + 0.2e1 * t1296 * t990;
t1300 = t51 * t13;
t1303 = t1258 * t1029;
t1304 = sin(epsRR_zs);
t1305 = t1304 * t5;
t1306 = t1305 * t7;
t1309 = t985 * t1121;
t1312 = I_wheel_yy * t22;
t1313 = t1312 * t987;
t1314 = t1121 * t5;
t1318 = t1312 * t995;
t1321 = r_wheelMntRL_Z * t5;
t1322 = t1321 * t7;
t1325 = t31 * t7;
t1329 = t1217 * t1029;
t1332 = r_wheelMntRL_X ^ 2;
t1336 = 2 * t3 * zRL_zs;
t1337 = t1074 * t996;
t1338 = I_body_zz * t1004;
t1342 = r_wheelMntRR_X ^ 2;
t1346 = -0.2e1 * t1300 * t1210 - 0.2e1 * t1303 * t1306 - 0.2e1 * t1309 * t1125 - 0.2e1 * t1313 * t1314 * t13 - 0.2e1 * t1318 * t1282 + 0.2e1 * t815 * t1322 - 0.2e1 * t1325 * t830 * t993 + 0.2e1 * t1329 * t1306 + t1138 * t1332 - t1034 * t993 + t1336 - t1337 + t1338 * t993 - 0.2e1 * t1003 * t993 + t1138 * t1342 - t994 * t1046 - t1059 * t993;
t1350 = t22 * zFL_zs;
t1352 = t22 * zFR_zs;
t1354 = I_body_yy * t7;
t1356 = I_body_zz * t7;
t1358 = t22 * zRR_zs;
t1360 = t22 * r_wheelMntRR_Z;
t1362 = I_wheel_yy * t13;
t1365 = t22 * r_wheelMntFR_Z;
t1367 = I_wheel_xx * t13;
t1370 = t22 * r_wheelMntRL_Z;
t1372 = t22 * zRL_zs;
t1374 = t18 * t1350 + t31 * t1352 + t1354 * t1154 - t1356 * t1154 + t25 * t1358 + t25 * t1360 + 0.2e1 * t1362 * t918 + t31 * t1365 - 0.4e1 * t1367 * t918 + t45 * t1370 + t45 * t1372;
t1375 = I_wheel_zz * t13;
t1378 = t22 * r_wheelMntFL_Z;
t1380 = r_wheelMntRL_X * zRL_zs;
t1381 = t1380 * t13;
t1383 = r_wheelMntRR_X * zRR_zs;
t1384 = t1383 * t13;
t1387 = t7 * t998;
t1390 = t1154 * t7;
t1393 = t22 * t988 * t1004;
t1396 = t22 * t1004;
t1405 = 0.2e1 * t1375 * t918 + t18 * t1378 - t787 * t1381 - t787 * t1384 + t1375 * t22 * t1387 * t996 + t1055 * t1390 - 0.2e1 * t1309 * t1393 - 0.2e1 * t3 * t1396 * r_wheelMntRL_Y + t1057 * t1390 - 0.2e1 * t16 * t1396 * r_wheelMntFR_Y + t1100 * t1390;
t1407 = t22 * t1039;
t1408 = t1407 * t1004;
t1411 = r_wheelMntFL_X * zFL_zs;
t1412 = t1411 * t13;
t1417 = r_wheelMntFR_X * r_wheelMntFR_Z;
t1418 = t1417 * t13;
t1427 = t1121 * t22;
t1428 = t1427 * t988;
t1430 = t1092 * t7;
t1431 = t1154 * t1002;
t1435 = I_wheel_yy * t5;
t1436 = t1145 * t7;
t1438 = 0.2e1 * t1038 * t1408 - t787 * t1412 - 0.2e1 * t18 * t1378 * t1004 - t787 * t1418 - 0.2e1 * t45 * t1372 * t1004 - 0.2e1 * t1169 * t1408 + 0.2e1 * t1122 * t1393 - t1120 * t1428 - t1430 * t1431 + 0.2e1 * t1092 * t1390 - t1435 * t1436;
t1439 = I_wheel_xx * t5;
t1441 = t995 * t7;
t1444 = I_wheel_zz * t5;
t1445 = t1029 * t1304;
t1446 = t1445 * t13;
t1453 = r_wheelMntRR_X * r_wheelMntRR_Y;
t1454 = t1453 * t7;
t1458 = t1037 * t22;
t1459 = t1458 * t1039;
t1464 = t29 * t22;
t1468 = t1439 * t1037 * t1441 * t998 + t1444 * t1446 - 0.2e1 * t31 * t1365 * t1004 - t1080 * t1390 + t1011 * t1390 + t787 * t1454 + t1103 * t1390 - t1034 * t1390 - t1036 * t1459 - 0.2e1 * t29 * t1396 * r_wheelMntFL_Y + 0.2e1 * t1464 * t788 * t13;
t1471 = t10 * t22;
t1475 = t1396 * r_wheelMntRR_Y;
t1478 = r_wheelMntFL_X * r_wheelMntFL_Y;
t1479 = t1478 * t7;
t1481 = t1018 * t13;
t1484 = t1014 * t7;
t1487 = t987 * t7;
t1492 = t989 * t13;
t1497 = r_wheelMntFR_X * zFR_zs;
t1498 = t1497 * t13;
t1500 = 0.2e1 * t1471 * t795 * t13 - 0.2e1 * t51 * t1475 + t787 * t1479 - t1481 * t918 * t996 + t1484 * t1431 - t1444 * t1121 * t1487 * t1013 + t1444 * t1436 - t1120 * t5 * t1492 - 0.2e1 * t1014 * t1390 - t1054 * t1390 - t787 * t1498;
t1504 = t1045 * t1225;
t1505 = t1504 * t13;
t1508 = t1121 * t7;
t1509 = t1508 * t1013;
t1511 = r_wheelMntRL_X * r_wheelMntRL_Z;
t1512 = t1511 * t13;
t1517 = t1076 * t7;
t1519 = r_wheelMntRL_X * r_wheelMntRL_Y;
t1520 = t1519 * t7;
t1522 = r_wheelMntFL_X * r_wheelMntFL_Z;
t1523 = t1522 * t13;
t1525 = -t1059 * t1390 + t1053 * t1390 - t1003 * t1390 - t1439 * t1505 + t1439 * t987 * t1509 - t787 * t1512 + 0.2e1 * t1018 * t1390 + t1049 * t1390 + t1444 * t1517 + t787 * t1520 - t787 * t1523;
t1532 = t1074 * t5;
t1537 = t1082 * t13;
t1539 = r_wheelMntRR_X * r_wheelMntRR_Z;
t1540 = t1539 * t13;
t1548 = t1109 * t1390 + t1168 * t1459 + t1367 * t918 * t1046 + t1187 * t1390 - t1532 * t1517 + t985 * t1428 - t1060 * t1390 + t1168 * t5 * t1537 - t787 * t1540 - 0.2e1 * t39 * t1475 + 0.2e1 * t39 * t22 * t801 * t13;
t1550 = t34 * t22;
t1551 = t805 * t13;
t1562 = r_wheelMntFR_X * r_wheelMntFR_Y;
t1563 = t1562 * t7;
t1570 = -t1022 * t1390 + 0.2e1 * t1550 * t1551 - t1439 * t1446 + t1184 * t1390 + t1008 * t1390 - t1051 * t1390 - t1435 * t1517 - 0.2e1 * t1375 * t918 * t998 + t787 * t1563 - t1036 * t5 * t1537 + t1444 * t1505 + t985 * t5 * t1492;
t1573 = t1374 + t1405 + t1438 + t1468 + t1500 + t1525 + t1548 + t1570;
t1574 = t1013 * t1002;
t1578 = t5 * zRR_zs;
t1585 = t918 * r_wheelMntFL_X;
t1589 = t989 * t7;
t1591 = t918 * r_wheelMntRL_X;
t1593 = t1145 * t13;
t1596 = t1445 * t7;
t1599 = -t1439 * t1574 - 0.2e1 * t3 * t1201 - 0.2e1 * t51 * t1578 - 0.2e1 * t16 * t1158 + t1444 * t1574 + t1444 * t999 - t49 * t1585 - t18 * t1154 * r_wheelMntFL_X + t986 * t1589 - t3 * t1591 - t1258 * t1593 - t34 * t1278 - t1217 * t1596 + t1312 * t1593;
t1600 = t1504 * t7;
t1605 = t1076 * t13;
t1607 = t1100 * t5;
t1608 = t1439 * t1046;
t1610 = t1055 * t5;
t1615 = t1057 * t5;
t1617 = t1258 * t1600 - t39 * t1116 - 0.2e1 * t1435 - t1439 * t999 - t1258 * t1605 - t1607 - t1608 - t1060 * t5 - t1610 + t1144 * t1593 - t1205 * t1593 + t1435 * t1002 + t1184 * t5 - t1615 + t1312 * t1605;
t1626 = t1018 * t22;
t1629 = t1082 * t7;
t1635 = t1444 * t1046;
t1636 = -t29 * t1585 - t25 * t1155 - t10 * t1591 - I_body_xx * t5 + t1075 * t1605 - t1296 * t1589 - t1217 * t1600 - t1626 * t1605 - t16 * t1278 + t1230 * t1629 - t51 * t1116 + t1258 * t1596 - t1081 * t1629 - 0.2e1 * t1444 + t1635;
t1637 = t1051 * t5;
t1638 = t1109 * t5;
t1639 = t1022 * t5;
t1640 = t1049 * t5;
t1641 = t1008 * t5;
t1642 = t1034 * t5;
t1643 = t1103 * t5;
t1644 = t1059 * t5;
t1650 = t1011 * t5;
t1651 = t1187 * t5;
t1653 = t1054 * t5;
t1654 = -t1637 - t1638 - t1639 - t1640 - t1641 - t1642 - t1643 - t1644 - 0.2e1 * t29 * t1233 - t45 * t1293 - t31 * t1154 * r_wheelMntFR_X - t1650 - t1651 - t1444 * t1002 + t1653;
t1656 = t1599 + t1617 + t1636 + t1654;
t1657 = m_wheel * t13;
t1659 = t18 * t5;
t1660 = -t1657 * t27 - t1659;
t1663 = -t1657 * t36 - t31 * t5;
t1665 = -t1657 * t43 - t1292;
t1667 = -t1657 * t23 - t1153;
t1668 = t987 * t13;
t1670 = I_wheel_yy * t1121;
t1672 = t1312 * t1668 - t1670 * t5;
t1673 = I_wheel_yy * t1037;
t1675 = t995 * t13;
t1677 = -t1673 * t5 + t1312 * t1675;
t1678 = t1312 * t13;
t1679 = M_FL;
t1682 = M_FR;
t1685 = t387 * r_DRL;
t1687 = M_RL;
t1691 = M_RR;
t1695 = I_wheel_zz * epsFR_zs1dot;
t1696 = t1695 * psi_zs1dot;
t1697 = t22 * t995;
t1698 = t1697 * t119;
t1701 = m_wheel * psi_zs1dot;
t1702 = t1701 * theta_zs1dot;
t1710 = t741 * r_DFR;
t1712 = t388 * r_DFR;
t1717 = psi_zs1dot * t1039;
t1718 = phi_zs1dot * t993;
t1719 = t1717 * t1718;
t1722 = t1074 * psi_zs1dot;
t1723 = theta_zs1dot * t995;
t1724 = t1037 * t13;
t1725 = t1723 * t1724;
t1729 = phi_zs1dot * psi_zs1dot;
t1730 = t1729 * t1124;
t1734 = t22 * t394;
t1736 = t29 * t133;
t1742 = t1145 * t867;
t1744 = t1082 * t871;
t1746 = t1710 * n_gndFR_X - t1712 * n_gndFR_Y - 0.2e1 * t1702 * t1539 * t7 - 0.2e1 * t1038 * t1719 + 0.2e1 * t1722 * t1725 + 0.2e1 * t1187 * t7 * t1730 - r_airRear_Z * t13 * t1734 + 0.4e1 * t1736 * t169 * t1096 + r_airRear_Y * t7 * t1734 - t1205 * t1742 - t1230 * t1744;
t1748 = t995 * epsFR_zs1dot;
t1749 = t1748 * t187;
t1755 = theta_zs1dot * phi_zs1dot;
t1759 = t133 * t987;
t1761 = t13 * t988;
t1762 = t1761 * epsFL_zs1dot;
t1763 = t1314 * t1762;
t1766 = I_wheel_xx * psi_zs1dot;
t1767 = t1766 * t998;
t1768 = t1041 * t174;
t1771 = t16 * t133;
t1772 = theta_zs1dot * t1004;
t1780 = t159 * t13;
t1784 = t211 * t13;
t1785 = r_wheelMntRL_Y * psi_zs1dot;
t1789 = t1103 * psi_zs1dot;
t1793 = t1049 * psi_zs1dot;
t1794 = t5 * t1004;
t1795 = t1794 * t228;
t1799 = t1729 * t1041;
t1802 = t123 * t13;
t1810 = I_wheel_zz * psi_zs1dot;
t1816 = t1755 * t1004;
t1820 = epsRR_zs1dot * t7 * phi_zs1dot;
t1824 = t1766 * t997;
t1825 = t1039 * epsFR_zs1dot;
t1826 = t1005 * t1825;
t1829 = t450 * zRR_zs;
t1831 = 0.2e1 * t1793 * t1795 - 0.2e1 * t1034 * t13 * t1799 + 0.2e1 * t1802 * t1352 * t169 + 0.2e1 * t1484 * t226 - t25 * t225 * r_wheelMntRR_Z - 0.4e1 * t1810 * t7 * t1025 * t174 + 0.2e1 * t1187 * t22 * t1816 + t1312 * t1820 + 0.4e1 * t1767 * t1795 + 0.4e1 * t1824 * t1826 + t1829 * t8;
t1834 = t1037 * psi_zs1dot;
t1835 = t1168 * t1834;
t1836 = t1004 * phi_zs1dot;
t1837 = t1039 * t993;
t1838 = t1836 * t1837;
t1841 = t1766 * theta_zs1dot;
t1848 = t148 * t22;
t1849 = t1848 * r_wheelMntRR_X;
t1851 = I_wheel_zz * epsFL_zs1dot;
t1853 = t1487 * phi_zs1dot;
t1855 = t51 * t133;
t1857 = r_wheelMntRR_Y * t5 * t13;
t1858 = t169 * t1857;
t1861 = t228 * phi_zs1dot;
t1865 = t174 * t23;
t1871 = t1439 * theta_zs1dot;
t1872 = t1030 * epsRR_zs1dot;
t1873 = t1872 * t13;
t1877 = t164 * r_wheelMntRR_Z;
t1878 = t1877 * t1004;
t1881 = t1039 * t7;
t1882 = t1723 * t1881;
t1888 = t22 * t1029;
t1890 = t1305 * t174;
t1893 = t1121 * psi_zs1dot;
t1894 = t1893 * t7;
t1896 = t22 * t5;
t1897 = t1896 * theta_zs1dot;
t1898 = t1761 * t1897;
t1906 = t13 * epsFR_zs1dot;
t1907 = t1906 * t1041;
t1910 = t1810 * t22;
t1911 = t1046 * epsRL_zs1dot;
t1912 = t1911 * t119;
t1915 = theta_zs1dot * t987;
t1916 = t1439 * t1915;
t1917 = t984 * t988;
t1918 = t1917 * epsFL_zs1dot;
t1922 = t1092 * psi_zs1dot;
t1925 = t22 * t987;
t1927 = t1121 * t13;
t1928 = phi_zs1dot * t988;
t1930 = t1927 * t1928 * epsFL_zs1dot;
t1933 = 0.2e1 * t1153 * t1878 - 0.2e1 * t1824 * t1882 + 0.2e1 * t1258 * t1030 * t1820 - 0.2e1 * t1766 * t1888 * t1890 - 0.4e1 * t1120 * t1894 * t1898 - 0.2e1 * t123 * zFR_zs * t5 * phi_zs1dot - 0.4e1 * t1074 * t1834 * t1907 - 0.4e1 * t1910 * t1912 - 0.2e1 * t1916 * t1508 * t1918 + 0.4e1 * t1922 * t1795 + 0.2e1 * t1120 * t1925 * t1930;
t1935 = t1120 * t918;
t1936 = t1002 * t988;
t1937 = t1936 * epsFL_zs1dot;
t1938 = t134 * t1937;
t1945 = t164 * t995;
t1946 = t1037 * t7;
t1954 = t29 * t187;
t1959 = I_wheel_xx * epsFL_zs1dot;
t1962 = t987 * epsFL_zs1dot;
t1963 = t1962 * t187;
t1969 = t792 * t164;
t1971 = t1258 * t164;
t1973 = 0.2e1 * t1935 * t1938 + 0.2e1 * t18 * t173 * t187 * t27 - t1075 * t1945 * t1946 - t1281 * t1946 * t148 + 0.2e1 * t1103 * t22 * t1816 + 0.4e1 * t1954 * r_wheelMntFL_Y * t22 * t134 + t1959 * t22 * t1853 + 0.2e1 * t1144 * t1963 - 0.2e1 * t1702 * t1411 * t7 + t1969 * t1454 + t1971 * t1446;
t1976 = theta_zs1dot * epsRR_zs1dot * t13;
t1978 = t1701 * t43;
t1982 = t3 * t22;
t1986 = t1092 * t1121;
t1987 = t228 * epsFL_zs1dot;
t1990 = t225 * t988;
t1993 = theta_zs1dot * epsRL_zs1dot * t13;
t1995 = t1003 * t1004;
t1998 = t854 * t13;
t2000 = t1092 * t133;
t2001 = t119 * phi_zs1dot;
t2002 = t1145 * t2001;
t2005 = t1504 * epsRL_zs1dot;
t2008 = -t1969 * t1412 - t1444 * t1976 - 0.2e1 * t1978 * t1201 * t174 - 0.4e1 * t1982 * t1755 * zRL_zs - 0.2e1 * t1986 * t1987 + t1122 * t1990 - t1435 * t1993 - 0.2e1 * t1995 * t1861 - t1638 * t1998 + 0.2e1 * t2000 * t2002 + 0.2e1 * t1810 * t2005;
t2012 = t51 * t22;
t2016 = psi_zs1dot * t993;
t2018 = t1145 * t134;
t2023 = epsRL_zs1dot * t7 * phi_zs1dot;
t2029 = t1375 * t228;
t2030 = t7 * t997;
t2031 = t996 * t1039;
t2032 = t2031 * epsFR_zs1dot;
t2033 = t2030 * t2032;
t2036 = zFR_zs * psi_zs1dot;
t2039 = I_wheel_xx * t1029;
t2041 = t1304 * epsRR_zs1dot;
t2042 = t169 * t2041;
t2046 = psi_zs1dot * t1004;
t2047 = t2046 * t993;
t2055 = t1074 * t133;
t2056 = t1748 * t119;
t2059 = t1014 * psi_zs1dot;
t2066 = t3 * psi_zs1dot;
t2067 = t169 * r_wheelMntRL_X;
t2070 = t989 * t871;
t2072 = t1014 * t1004;
t2077 = t1225 * t13;
t2078 = t2077 * t148;
t2080 = I_wheel_yy * epsFL_zs1dot;
t2081 = t2080 * t5;
t2082 = t1915 * t13;
t2089 = t387 * t4;
t2091 = -0.4e1 * t2055 * t2056 + 0.2e1 * t2059 * t1897 + 0.4e1 * t45 * t173 * t822 * t267 - 0.2e1 * t2066 * t2067 - t986 * t2070 - 0.4e1 * t2072 * t1861 - 0.2e1 * t1205 * t1963 + t1224 * t2078 - t2081 * t2082 + 0.2e1 * t1766 * t1697 * t1219 * t187 * t998 + t2089 * t43;
t2093 = t1370 * t169;
t2098 = t644 * zRR_zs;
t2100 = t1766 * t22;
t2104 = t1028 * t1030;
t2107 = I_wheel_yy * psi_zs1dot;
t2108 = t2107 * t993;
t2109 = t7 * t13;
t2110 = t2109 * phi_zs1dot;
t2113 = t1217 * t164;
t2116 = t1701 * t5;
t2121 = theta_zs1dot * t1037;
t2122 = t1439 * t2121;
t2123 = t997 * t1039;
t2124 = t2123 * epsFR_zs1dot;
t2129 = t1014 * t133;
t2132 = 0.2e1 * t1784 * t2093 - 0.2e1 * t1430 * t226 - t2098 * t96 + 0.4e1 * t2100 * t999 * t293 + 0.2e1 * t2104 * t1861 + 0.4e1 * t2108 * t2110 + t2113 * t1076 * t1387 - 0.2e1 * t2116 * theta_zs1dot * t1342 * t22 - 0.2e1 * t2122 * t1441 * t2124 - t1607 * t1998 - 0.2e1 * t2129 * t2002;
t2133 = t1444 * phi_zs1dot;
t2134 = t997 * t996;
t2135 = t2134 * t1825;
t2139 = phi_zs1dot * r_wheelMntFL_Z;
t2143 = t985 * psi_zs1dot;
t2144 = t988 * epsFL_zs1dot;
t2145 = t1005 * t2144;
t2150 = t1015 * t2144;
t2153 = t388 * zFR_zs;
t2155 = t1837 * epsFR_zs1dot;
t2163 = t7 * epsFL_zs1dot;
t2164 = t2163 * t1124;
t2167 = t1766 * t1004;
t2168 = t22 * t1030;
t2172 = t1834 * t13;
t2174 = t1881 * t1897;
t2177 = -0.2e1 * t2133 * t2135 + 0.4e1 * t29 * t139 * t2139 * t1041 - 0.4e1 * t2143 * t2145 - 0.2e1 * t1767 * t1897 - 0.4e1 * t2143 * t2150 - t2153 * t14 - 0.2e1 * t1824 * t2155 + 0.4e1 * t18 * t133 * t134 * t1234 - 0.4e1 * t1014 * t1893 * t2164 + 0.2e1 * t2167 * t2168 * t293 - 0.4e1 * t1036 * t2172 * t2174;
t2180 = t388 * r_wheelMntFR_Z;
t2182 = t25 * phi_zs1dot;
t2183 = r_wheelMntRR_Z * psi_zs1dot;
t2190 = t1034 * psi_zs1dot;
t2193 = t2107 * t1002;
t2197 = t993 * t1029;
t2201 = t1011 * psi_zs1dot;
t2204 = t1002 * t22;
t2205 = t2204 * t293;
t2209 = t984 * t1002 * t2144;
t2213 = t1018 * t1004;
t2216 = t644 * r_wheelMntRR_Y;
t2220 = t174 * t27;
t2223 = t669 * zRL_zs;
t2228 = t261 * t13;
t2229 = r_wheelMntRR_Y * psi_zs1dot;
t2233 = t669 * r_wheelMntRL_Z;
t2239 = phi_zs1dot * t1039;
t2241 = t1724 * t2239 * epsFR_zs1dot;
t2244 = t565 * r_wheelMntFL_Y;
t2246 = 0.4e1 * t2213 * t1861 - t2216 * t93 + t1356 * t226 - 0.2e1 * t49 * t173 * t2220 - t2223 * t90 + 0.4e1 * t1018 * t1834 * t1907 - 0.2e1 * t2228 * t2229 * t1041 - t2233 * t96 - 0.4e1 * t1168 * t2016 * t1882 - 0.2e1 * t1168 * t1697 * t2241 + t2244 * t87;
t2248 = t1810 * theta_zs1dot;
t2251 = t1766 * t7;
t2258 = t1028 * t1013;
t2261 = I_body_yy * psi_zs1dot;
t2263 = t1794 * theta_zs1dot;
t2266 = t34 * t5;
t2271 = t164 * t987 * t1761;
t2276 = t1962 * t119;
t2279 = t1076 * t867;
t2281 = -0.2e1 * t2248 * t1593 + 0.2e1 * t2251 * t1031 * t174 + 0.4e1 * t1036 * t1834 * t1838 + 0.4e1 * t2258 * t1861 + 0.2e1 * t2261 * t22 * t2263 - 0.2e1 * t2266 * t854 * t824 - t1296 * t2271 - 0.2e1 * t1338 * t1861 - t1258 * t2023 + 0.4e1 * t2000 * t2276 + t1075 * t2279;
t2287 = t1219 * t187;
t2300 = phi_zs1dot * t22;
t2304 = phi_zs1dot * t1002;
t2305 = t228 * t2304;
t2308 = t1766 * t993;
t2316 = t1060 * t7 * t226 + 0.4e1 * t1922 * t2205 + 0.2e1 * t1810 * t1697 * t2287 - 0.4e1 * t2108 * t2018 - 0.8e1 * t1028 * t1861 - 0.4e1 * t1766 * t1697 * t1037 * t181 * t2124 - 0.2e1 * t159 * t7 * t2300 * r_wheelMntFL_X + 0.2e1 * t2072 * t2305 + 0.4e1 * t2308 * t2135 + t1144 * t1742 - 0.2e1 * t29 * t5 * t854 * t818;
t2321 = t1810 * t997;
t2324 = t1848 * r_wheelMntFR_X;
t2326 = t164 * t1004;
t2327 = t2326 * r_wheelMntFR_Y;
t2335 = t1024 * t1030;
t2341 = t1060 * t1004;
t2344 = t1458 * theta_zs1dot;
t2347 = t228 * t1046;
t2351 = I_wheel_xx * epsFR_zs1dot;
t2352 = t2351 * psi_zs1dot;
t2356 = t2080 * t22;
t2362 = t669 * t12;
t2371 = t565 * r_wheelMntFL_Z;
t2373 = t1092 * t5;
t2374 = epsFL_zs1dot * t13;
t2375 = t1915 * t2374;
t2381 = t1444 * theta_zs1dot * t1121;
t2385 = -0.2e1 * t2352 * t1698 - t2233 * t90 + t2356 * t1853 - 0.2e1 * t2107 * t1925 * t1314 * t187 - t2362 * t43 - 0.2e1 * t261 * t1578 * phi_zs1dot + 0.4e1 * t1910 * t996 * t5 * theta_zs1dot - t2371 * t90 - 0.2e1 * t2373 * t2375 - 0.4e1 * t2108 * t1725 + 0.2e1 * t2381 * t1487 * t1918;
t2390 = t10 * t187;
t2391 = r_wheelMntRL_Z * psi_zs1dot;
t2397 = t1120 * psi_zs1dot;
t2400 = t2107 * t22;
t2418 = t450 * r_wheelMntRR_Y;
t2425 = t261 * psi_zs1dot;
t2428 = t1427 * theta_zs1dot;
t2432 = t7 * t996;
t2435 = t1810 * t1004;
t2436 = t997 * t993;
t2441 = t1046 * t5;
t2442 = t2441 * theta_zs1dot;
t2449 = t1439 * phi_zs1dot;
t2452 = 0.2e1 * t1722 * t1897 + t16 * t13 * t2324 - 0.2e1 * t2425 * t1214 - t2080 * t2428 + 0.4e1 * t1024 * t1861 + t1481 * t225 * t2432 - 0.4e1 * t2435 * t2436 * t1825 - t1626 * t2279 - 0.2e1 * t1910 * t2442 - 0.2e1 * t261 * t7 * t2300 * r_wheelMntRR_X + 0.2e1 * t2449 * t2135;
t2456 = t669 * r_wheelMntRL_Y;
t2458 = t1051 * psi_zs1dot;
t2465 = t998 * t22;
t2470 = t1039 * t1004;
t2471 = t225 * t2470;
t2474 = t387 * zRL_zs;
t2476 = I_wheel_zz * t1029;
t2481 = t1168 * t133;
t2482 = t1082 * t213;
t2486 = epsRL_zs1dot * t5 * t7;
t2489 = t246 * t4;
t2491 = t1766 * t999;
t2497 = t1810 * t996;
t2500 = t1008 * psi_zs1dot;
t2505 = t10 * t173;
t2506 = t228 * t13;
t2511 = epsRR_zs1dot * t5 * t7;
t2514 = 0.2e1 * t2481 * t2482 + 0.2e1 * t1910 * t2486 + t2489 * t27 - 0.2e1 * t2491 * t1768 - 0.2e1 * t2458 * t1795 - t2456 * t93 - 0.2e1 * t2497 * t1795 + 0.2e1 * t2500 * t1768 - 0.2e1 * t1824 * t2032 + 0.4e1 * t2505 * t836 * t2506 - 0.2e1 * t2100 * t2511;
t2517 = t989 * t169;
t2529 = t1810 * t993;
t2535 = t1851 * t1121;
t2536 = t228 * t1004;
t2540 = r_wheelMntFR_Z * psi_zs1dot;
t2544 = t1004 * t988;
t2545 = t2544 * t1718;
t2548 = t387 * r_wheelMntRL_Y;
t2550 = 0.4e1 * t1120 * t2016 * t2517 - t1367 * t5 * t854 * t1046 + 0.2e1 * t2261 * t993 * t2110 - 0.2e1 * t123 * t1158 * phi_zs1dot - 0.2e1 * t2529 * t2005 + 0.2e1 * t1011 * t7 * t1730 + 0.2e1 * t2535 * t2536 - t1969 * t1540 + 0.2e1 * t123 * t2540 + 0.4e1 * t1120 * t1893 * t2545 + t2548 * t32;
t2553 = t1120 * t133;
t2554 = t989 * t213;
t2557 = t1018 * t1037;
t2559 = t228 * epsFR_zs1dot * t1004;
t2564 = phi_zs1dot * t1304 * epsRR_zs1dot;
t2568 = t1810 * t999;
t2572 = t388 * t4;
t2578 = t387 * r_wheelMntRL_Z;
t2580 = t1054 * t13 * t232 - 0.2e1 * t2553 * t2554 + 0.4e1 * t2557 * t2559 + 0.2e1 * t2039 * t5 * t2564 + t1439 * t1976 + 0.2e1 * t2568 * t1768 - t1969 * t1512 + t2572 * t36 + t1312 * t1037 * t1441 * t148 + t2548 * t19 + t2578 * t8;
t2584 = t246 * zFL_zs;
t2586 = t1445 * epsRR_zs1dot;
t2589 = t741 * zFR_zs;
t2596 = t1365 * t169;
t2600 = t246 * r_wheelMntFL_Y;
t2604 = t993 * t995;
t2610 = t2030 * t1825;
t2619 = t1695 * t5;
t2620 = t1723 * t13;
t2622 = t1360 * t169;
t2625 = t741 * r_wheelMntFR_Y;
t2627 = t1018 * t5;
t2628 = t1723 * t1906;
t2633 = t2107 * theta_zs1dot;
t2636 = t644 * t12;
t2641 = 0.4e1 * t2029 * t2610 - 0.2e1 * t211 * t22 * t1772 * r_wheelMntRL_Y - t45 * t225 * zRL_zs - t2619 * t2620 + 0.2e1 * t2228 * t2622 - t2625 * t93 - 0.2e1 * t2627 * t2628 - t18 * t225 * zFL_zs + 0.2e1 * t2633 * t1593 - t2636 * t23 + 0.2e1 * t1100 * t22 * t1816;
t2647 = t39 * t187;
t2651 = t741 * r_wheelMntFR_Z;
t2657 = t1054 * psi_zs1dot;
t2660 = t246 * r_wheelMntFL_Z;
t2664 = t1076 * t1220;
t2670 = 0.4e1 * t1702 * t1562 * t1124 + t1971 * t1436 + 0.4e1 * t2647 * t2183 * t1124 - t2651 * t96 + 0.2e1 * t2449 * t2209 - 0.2e1 * t2397 * t1937 - 0.2e1 * t2657 * t1795 + t2660 * t8 + 0.2e1 * t1169 * t2471 - 0.2e1 * t1841 * t2664 + 0.2e1 * t1258 * t1046 * t2023;
t2671 = t565 * t12;
t2675 = t2107 * t996;
t2678 = psi_zs1dot * t1002;
t2679 = t1092 * t2678;
t2682 = t1504 * t169;
t2688 = t993 * t988;
t2689 = t2688 * epsFL_zs1dot;
t2692 = t388 * r_wheelMntFR_Y;
t2694 = t1003 * psi_zs1dot;
t2700 = t565 * zFL_zs;
t2702 = -t2671 * t27 - 0.2e1 * t1055 * t1861 - 0.4e1 * t2675 * t1897 - 0.2e1 * t2679 * t1768 - 0.4e1 * t2529 * t2682 - 0.2e1 * t1702 * t1417 * t7 + 0.2e1 * t2143 * t2689 + t2692 * t19 - 0.2e1 * t2694 * t1795 - 0.2e1 * t2055 * t1076 * t2001 - t2700 * t90;
t2707 = t1014 * t5;
t2711 = t1848 * r_wheelMntRL_X;
t2717 = t1848 * r_wheelMntFL_X;
t2719 = t644 * r_wheelMntRR_Z;
t2727 = t31 * t174;
t2742 = t39 * psi_zs1dot;
t2743 = phi_zs1dot * r_wheelMntRR_Y;
t2747 = t1036 * t1458;
t2748 = theta_zs1dot * t1039;
t2766 = 0.4e1 * t2647 * r_wheelMntRR_Y * t22 * t134 + 0.4e1 * t1702 * t1417 * t1041 - t2584 * t14 + 0.2e1 * t2742 * t2743 * t993 - 0.4e1 * t2747 * t2748 * t2110 - t1969 * t1498 - t1829 * t14 - 0.2e1 * t261 * r_wheelMntRR_Z * t5 * phi_zs1dot - 0.2e1 * t1051 * t13 * t1799 - 0.4e1 * t2742 * t2743 * t1005 - 0.2e1 * t1375 * t232;
t2768 = t2476 * psi_zs1dot;
t2772 = t13 * t1002;
t2773 = t225 * t2772;
t2779 = I_wheel_zz * t1045;
t2781 = t1225 * epsRL_zs1dot;
t2786 = t2351 * t1037;
t2789 = t225 * t2544;
t2796 = -0.2e1 * t2768 * t1005 * t2041 - t1484 * t2773 - t1289 * t2078 + t1644 * t1998 + t1003 * t7 * t226 + 0.2e1 * t2779 * t1154 * t169 * t2781 + t1217 * t2023 - 0.2e1 * t2786 * t2536 + 0.2e1 * t1309 * t2789 + 0.2e1 * t2633 * t1605 + 0.2e1 * t1793 * t1768;
t2808 = t1100 * psi_zs1dot;
t2811 = t1024 * t1046;
t2815 = t1034 * t22;
t2820 = t16 * psi_zs1dot;
t2821 = phi_zs1dot * r_wheelMntFR_Y;
t2825 = -0.2e1 * t1022 * t22 * t1816 + 0.2e1 * t2193 * t1795 + t1969 * t1479 - 0.2e1 * t1217 * t1030 * t1820 - 0.2e1 * t2657 * t1768 + 0.2e1 * t2808 * t1795 - 0.2e1 * t2811 * t1861 + t2418 * t19 - 0.2e1 * t2815 * t1816 - 0.2e1 * t1092 * t1861 - 0.4e1 * t2820 * t2821 * t1005;
t2832 = I_wheel_xx * t1045;
t2834 = t1005 * t2781;
t2837 = t1024 * phi_zs1dot;
t2838 = t228 * t998;
t2841 = t18 * phi_zs1dot;
t2842 = zFL_zs * psi_zs1dot;
t2848 = t450 * t4;
t2853 = t134 * t2144;
t2856 = t1755 * t1046;
t2860 = t164 * zFL_zs;
t2861 = t2860 * t1004;
t2864 = I_body_zz * psi_zs1dot;
t2873 = t1695 * t1037;
t2877 = t3 * t5;
t2878 = t2326 * r_wheelMntRL_Y;
t2881 = t45 * psi_zs1dot;
t2882 = t134 * r_wheelMntRL_X;
t2888 = t1047 * psi_zs1dot;
t2891 = 0.2e1 * t1659 * t2861 - 0.2e1 * t2864 * t1004 * t1897 + t2216 * t87 + 0.4e1 * t2308 * t2682 + 0.2e1 * t2449 * t2005 + 0.2e1 * t2873 * t2536 + t1637 * t1998 + 0.2e1 * t2877 * t2878 - 0.2e1 * t2881 * t2882 + 0.4e1 * t1092 * t1893 * t2164 + 0.2e1 * t2888 * t1768;
t2893 = t1124 * phi_zs1dot;
t2898 = t16 * t187;
t2902 = r_wheelMntFR_Y * t22;
t2907 = I_wheel_yy * epsFR_zs1dot;
t2908 = t2907 * t5;
t2915 = t1040 * epsFR_zs1dot;
t2921 = t1304 * t13;
t2922 = t2921 * t148;
t2926 = t1959 * t5;
t2943 = t1036 * t133;
t2949 = t1312 * t2023 + t2926 * t2082 - 0.2e1 * t29 * t173 * t2220 - t45 * t225 * r_wheelMntRL_Z - t1615 * t1998 + 0.4e1 * t1036 * t2016 * t1882 - 0.2e1 * t261 * t22 * t1772 * r_wheelMntRR_Y - t1184 * t7 * t226 - 0.2e1 * t2943 * t2482 + t1209 * t1849 - 0.2e1 * t2694 * t1768;
t2957 = t22 * t1045;
t2959 = t1226 * t174;
t2962 = t1851 * psi_zs1dot;
t2963 = t1925 * t119;
t2982 = t450 * r_wheelMntRR_Z;
t2991 = zRL_zs * phi_zs1dot;
t3001 = 0.2e1 * t2321 * t1882 - t2371 * t96 + 0.2e1 * t1810 * t2134 * t1826 + t1430 * t2773 + t2982 * t8 - 0.2e1 * t2133 * t2005 + 0.4e1 * t1217 * t1755 + 0.2e1 * t985 * t2678 * t2145 + 0.2e1 * t2881 * t2991 * t993 - 0.2e1 * t1810 * t1045 * t2834 + 0.4e1 * t1092 * t2016 * t2018;
t3003 = t2907 * t22;
t3004 = t1441 * phi_zs1dot;
t3009 = t1810 * t1046;
t3013 = t174 * t36;
t3016 = t123 * psi_zs1dot;
t3027 = t18 * t174;
t3028 = t1378 * t169;
t3031 = t3003 * t3004 - 0.2e1 * t1362 * t232 + t1329 * t2922 - 0.2e1 * t3009 * t1768 - 0.2e1 * t34 * t173 * t3013 - 0.2e1 * t3016 * t826 * t1124 + 0.2e1 * t2675 * t1795 - t1354 * t226 + 0.2e1 * t2500 * t1795 + 0.4e1 * t2529 * t2110 + 0.4e1 * t3027 * t3028;
t3034 = t31 * phi_zs1dot;
t3049 = t1004 * r_wheelMntRL_Z;
t3053 = t1478 * t13;
t3056 = t31 * t133;
t3062 = -0.2e1 * t3009 * t1795 - 0.4e1 * t3034 * t2540 * t1005 - t25 * t225 * zRR_zs + 0.2e1 * t1810 * t2957 * t2959 + 0.2e1 * t2568 * t1795 + 0.2e1 * t211 * t2391 - 0.2e1 * t1011 * t1861 + 0.4e1 * t2505 * t3049 * t228 - 0.2e1 * t1702 * t3053 + 0.4e1 * t3056 * t134 * t1159 - 0.2e1 * t3016 * t1133;
t3066 = t1184 * t1004;
t3069 = t1945 * t1040;
t3071 = t10 * psi_zs1dot;
t3072 = t1004 * r_wheelMntRL_Y;
t3073 = t3072 * t1718;
t3078 = t565 * r_DFL;
t3082 = t1014 * t2678;
t3085 = t152 * t1124;
t3089 = t134 * phi_zs1dot;
t3102 = r_wheelMntFL_Z * psi_zs1dot;
t3106 = t1872 * t119;
t3109 = t1074 * t1037;
t3117 = t159 * psi_zs1dot;
t3118 = t1004 * r_wheelMntFL_Z;
t3119 = t3118 * t993;
t3124 = 0.2e1 * t1011 * t22 * t1816 + 0.2e1 * t1169 * t1719 - 0.2e1 * t2258 * t2305 - 0.4e1 * t2841 * t3102 * t1005 - 0.4e1 * t1910 * t3106 - 0.4e1 * t3109 * t2559 + 0.2e1 * t1014 * t1861 - t2098 * t90 - 0.2e1 * t1922 * t2018 - 0.2e1 * t3117 * t3119 - t1053 * t7 * t226;
t3126 = zRR_zs * psi_zs1dot;
t3129 = t1445 * t169;
t3145 = t1030 * t5;
t3146 = t3145 * theta_zs1dot;
t3157 = zRL_zs * psi_zs1dot;
t3160 = 0.2e1 * t261 * t3126 - 0.4e1 * t2529 * t3129 + 0.4e1 * t1550 * t1755 * zFR_zs * t1004 - 0.2e1 * t2832 * psi_zs1dot * t1225 * epsRL_zs1dot + 0.2e1 * t2675 * t1768 - 0.2e1 * t2877 * t854 * t834 + 0.2e1 * t2100 * t3146 - 0.2e1 * t211 * t1321 * phi_zs1dot - 0.2e1 * t1766 * t2134 * t1826 + 0.2e1 * t2873 * t3085 + 0.2e1 * t211 * t3157;
t3161 = t993 * theta_zs1dot;
t3162 = t7 * r_wheelMntRR_X;
t3163 = t3161 * t3162;
t3171 = t1022 * psi_zs1dot;
t3187 = 0.4e1 * t2742 * t3163 - t2589 * t90 + 0.2e1 * t2808 * t1768 + 0.4e1 * t1910 * t2263 + 0.2e1 * t3171 * t1897 - 0.2e1 * t3117 * t1267 + 0.4e1 * t1018 * t133 * t2056 - t1695 * t22 * t3004 + 0.2e1 * t1780 * t3028 + 0.2e1 * t261 * t2183 - 0.2e1 * t1187 * t1861;
t3195 = t1014 * t1121;
t3197 = t228 * epsFL_zs1dot * t1004;
t3211 = t164 * zRR_zs;
t3220 = I_body_yy * t1004;
t3223 = t1701 * t993;
t3227 = t225 * t1039;
t3244 = 0.2e1 * t1910 * t2511 + 0.2e1 * t3220 * t1861 + 0.4e1 * t3223 * t1380 * t169 + t1038 * t3227 + 0.2e1 * t49 * t5 * t2326 * r_wheelMntFL_Y - t2113 * t1446 - 0.4e1 * t1258 * t1755 + 0.4e1 * t1986 * t3197 - 0.2e1 * t16 * t173 * t3013 - 0.2e1 * t2397 * t2689 + t1296 * t2070;
t3247 = t228 * epsFR_zs1dot;
t3254 = t1057 * psi_zs1dot;
t3259 = t1120 * t1427;
t3260 = theta_zs1dot * t988;
t3261 = t3260 * t2110;
t3264 = t25 * t174;
t3267 = t1444 * theta_zs1dot;
t3279 = t2625 * t87 - 0.2e1 * t2557 * t3247 + 0.2e1 * t25 * t173 * t187 * t23 + 0.2e1 * t3254 * t1768 + 0.2e1 * t2248 * t1596 - 0.4e1 * t3259 * t3261 + 0.4e1 * t3264 * t2622 + 0.2e1 * t3267 * t1873 - 0.2e1 * t3117 * t840 * t1124 + 0.4e1 * t2881 * t134 * r_wheelMntRL_X * t993 + 0.4e1 * t2397 * t2145;
t3296 = t1109 * t22;
t3304 = t741 * t12;
t3306 = t34 * t13 * t2324 - 0.2e1 * t1109 * t1861 - t1969 * t1523 - 0.2e1 * t211 * t1201 * phi_zs1dot - 0.2e1 * t159 * t1164 * phi_zs1dot + 0.4e1 * t2400 * t2263 + t22 * r_airFront_X * t341 * t13 + 0.2e1 * t3296 * t1816 + t2351 * t22 * t3004 - 0.2e1 * t1270 * t854 * t828 - t3304 * t36;
t3311 = t7 * t1013;
t3312 = t1145 * t3311;
t3339 = t1053 * t1004;
t3353 = t1375 * t5;
t3359 = t985 * t918;
t3362 = -t1969 * t1418 + 0.2e1 * t2059 * t2018 + 0.2e1 * t2266 * t2327 + 0.2e1 * t3339 * t1861 + 0.2e1 * t1784 * t1372 * t169 + 0.2e1 * t1978 * r_wheelMntRL_Y * t5 * t187 + t1067 * t2717 + 0.4e1 * t3223 * t1511 * t169 + 0.2e1 * t3353 * t854 * t998 - 0.2e1 * t1922 * t1897 - 0.2e1 * t3359 * t1938;
t3364 = t1959 * t1121;
t3367 = t985 * t1427;
t3370 = t1312 * t164;
t3387 = t51 * psi_zs1dot;
t3407 = I_wheel_yy * t1004;
t3414 = -t2907 * t2344 + 0.4e1 * t3387 * t3163 - 0.2e1 * t1978 * t1321 * t174 + 0.2e1 * t2190 * t1897 - 0.2e1 * t2864 * t7 * t2893 - 0.2e1 * t123 * zFR_zs * t2047 - 0.2e1 * t123 * t7 * t2300 * r_wheelMntFR_X + 0.4e1 * t2694 * t1897 + 0.4e1 * t3407 * t1861 - 0.2e1 * t159 * t1233 * phi_zs1dot + t1300 * t1849;
t3418 = t22 * t454;
t3420 = t18 * psi_zs1dot;
t3421 = t13 * r_wheelMntFL_X;
t3428 = t1168 * t293;
t3429 = t1881 * epsFR_zs1dot;
t3453 = t7 * r_wheelMntFR_X;
t3458 = t1701 * t22;
t3465 = t7 * t1045 * t2781;
t3472 = -t1640 * t1998 + 0.4e1 * t39 * t133 * t1858 - 0.2e1 * t2397 * t2517 + t2113 * t3312 - 0.4e1 * t2066 * t3073 + 0.4e1 * t2820 * t3161 * t3453 - t1309 * t1990 + 0.2e1 * t3458 * r_wheelMntRL_X * zRL_zs1dot * t119 - 0.2e1 * t1367 * t228 * t3465 - 0.2e1 * t1841 * t1600 + r_airFront_Y * t7 * t3418;
t3476 = I_body_xx * phi_zs1dot;
t3480 = r_wheelMntRL_Y * t22;
t3484 = t1059 * psi_zs1dot;
t3487 = t1959 * psi_zs1dot;
t3497 = t2351 * t2344 + t1969 * t1563 - t3476 * t228 + 0.2e1 * t2308 * t2586 + 0.4e1 * t2390 * t3480 * t134 + 0.2e1 * t3484 * t1897 - 0.2e1 * t3487 * t2963 - t2578 * t14 - 0.4e1 * t2059 * t1795 - 0.2e1 * t211 * zRL_zs * t2047 - t1169 * t3227;
t3504 = r_wheelMntRL_Z * phi_zs1dot;
t3517 = t228 * t999;
t3529 = 0.2e1 * t1109 * psi_zs1dot * t1795 + 0.2e1 * t2425 * t119 * t23 + 0.2e1 * t2881 * t3504 * t993 + 0.2e1 * t2476 * psi_zs1dot * t1304 * epsRR_zs1dot - 0.2e1 * t3484 * t1795 + t1642 * t1998 - 0.4e1 * t2059 * t1768 + 0.2e1 * t2837 * t3517 + 0.2e1 * t2841 * t3102 * t993 + 0.4e1 * t2100 * t3106 - 0.2e1 * t211 * t7 * t2300 * r_wheelMntRL_X;
t3533 = I_wheel_yy * phi_zs1dot;
t3548 = t22 * t996;
t3552 = t450 * r_DRR;
t3568 = t45 * t174;
t3571 = t1851 * t5;
t3573 = t1729 * t2688;
t3576 = I_body_xx * psi_zs1dot;
t3579 = t29 * psi_zs1dot;
t3580 = t7 * r_wheelMntFL_X;
t3586 = 0.2e1 * t2143 * t2517 + 0.2e1 * t3195 * t1987 - 0.2e1 * t1702 * t1497 * t7 + 0.4e1 * t2529 * t2018 + t1971 * t1505 + 0.4e1 * t3568 * t2093 - t3571 * t2082 - 0.2e1 * t1122 * t3573 + 0.2e1 * t3576 * t1897 + 0.4e1 * t3579 * t3161 * t3580 + 0.4e1 * t2308 * t3129;
t3591 = t644 * r_DRR;
t3610 = t1911 * t13;
t3613 = -0.2e1 * t1059 * t13 * t1799 + t3591 * n_gndRR_X - t3353 * t854 * t999 - t1641 * t1998 - 0.2e1 * t1059 * t22 * t1816 - 0.2e1 * t1057 * t1861 - 0.2e1 * t2248 * t1605 + 0.2e1 * t1054 * t1861 - 0.4e1 * t2321 * t1071 * t1825 - 0.2e1 * t1018 * t1861 + 0.2e1 * t3267 * t3610;
t3614 = t985 * t133;
t3642 = 0.2e1 * t3614 * t2554 - t2982 * t14 + 0.2e1 * t159 * t3102 + 0.2e1 * t2321 * t2032 - 0.2e1 * t2116 * theta_zs1dot * t1264 * t22 + 0.2e1 * t3016 * t119 * t36 + t1313 * t1508 * t148 - 0.2e1 * t3458 * t1332 * t5 * theta_zs1dot - 0.4e1 * t2129 * t2276 - 0.2e1 * t2786 * t3085 + 0.2e1 * t2820 * t2821 * t993;
t3647 = t1036 * t1154;
t3651 = t2351 * t5;
t3659 = t1522 * t7;
t3683 = t1049 * t22;
t3694 = -t1055 * t13 * t232 - 0.2e1 * t1910 * t3146 + 0.2e1 * t1810 * t1427 * t1260 * t187 - 0.2e1 * t3171 * t1768 + 0.2e1 * t2182 * t2183 * t993 - t1086 * t2711 + 0.2e1 * t3683 * t1816 - I_body_yy * phi_zs1dot * t228 - t1259 * t1487 * t148 + t2600 * t19 + 0.2e1 * t3647 * t169 * t2032;
t3700 = theta_zs1dot * t996;
t3713 = t1187 * psi_zs1dot;
t3720 = -t1969 * t1384 + 0.2e1 * t1309 * t3573 - t2651 * t90 - 0.2e1 * t2213 * t2300 * t3700 + 0.4e1 * t1982 * t1755 * t1104 + 0.4e1 * t1736 * t1772 * t1233 + 0.2e1 * t10 * t5 * t2878 + 0.2e1 * t3713 * t1795 + 0.4e1 * t2529 * t1725 - t2700 * t96 - t1643 * t1998;
t3728 = t29 * t1004;
t3729 = phi_zs1dot * r_wheelMntFL_Y;
t3743 = t669 * r_DRL;
t3745 = t246 * r_DFL;
t3747 = 0.2e1 * t1258 * t1755 * t998 - 0.2e1 * t3071 * t2067 - 0.2e1 * t2529 * t2586 - 0.4e1 * t3728 * t3729 * t2016 + 0.2e1 * t2308 * t2005 - t1650 * t1998 - 0.2e1 * t3364 * t2536 - 0.2e1 * t261 * r_wheelMntRR_Z * t2047 - 0.2e1 * t1871 * t3610 + t3743 * n_gndRL_X - t3745 * n_gndFL_Y;
t3754 = t996 * t1004;
t3756 = m_wheel * t1004;
t3760 = t1002 * t1004;
t3766 = t3756 * t1007;
t3768 = t1508 * t988;
t3771 = m_wheel * t7;
t3776 = t3756 * t1099;
t3777 = t3756 * t1108;
t3782 = t1074 + t1074 * t3754 + 0.2e1 * t3756 * zRR_zs * r_wheelMntRR_Z - t1092 * t3760 + t1014 * t3760 + 0.2e1 * t3756 * zFL_zs * r_wheelMntFL_Z + t3766 - 0.2e1 * t1120 * t13 * t3768 + 0.2e1 * t3771 * t834 * r_wheelMntRL_Y + 0.2e1 * t2258 + t3776 + t3777 + 0.2e1 * t3771 * t820 * r_wheelMntRR_Y - 0.2e1 * t2072 - t1995 + t3339;
t3783 = t3756 * t1102;
t3785 = t3756 * t1048;
t3795 = t3783 - t1018 * t3754 + t3785 - t1047 + t1051 + 0.2e1 * t3756 * zRL_zs * r_wheelMntRL_Z - t1338 - t1092 + t3220 - t2335 + m_wheel * t1332 + 0.2e1 * t3756 * zFR_zs * r_wheelMntFR_Z + t1022 + m_wheel * t1342 + m_wheel * t1139 + t1054 - t1055;
t3814 = -0.4e1 * t1028 + t3066 + m_wheel * t1264 + t1059 - t2341 - t1018 - 0.2e1 * t1024 * t998 + t1080 + 0.2e1 * t2213 - t2811 + 0.2e1 * t1024 + 0.2e1 * t3407 + 0.2e1 * t3771 * t838 * r_wheelMntFL_Y + t1028 * t1046 + 0.2e1 * t3771 * t824 * r_wheelMntFR_Y + 0.2e1 * t1657 * t832 * r_wheelMntRR_Z + t2104;
t3823 = t3756 * t1010;
t3824 = t3756 * t1186;
t3827 = t1946 * t1039;
t3831 = t3756 * t1056;
t3842 = -t1051 * t1004 + 0.2e1 * t985 * t13 * t3768 + t1034 + 0.2e1 * t1657 * t836 * r_wheelMntRL_Z + t1014 - t1034 * t1004 + t3823 + t3824 - t1022 * t1004 + 0.2e1 * t1168 * t13 * t3827 - t1059 * t1004 + t3831 + 0.4e1 * I_wheel_xx + 0.2e1 * t1657 * t826 * r_wheelMntFR_Z - 0.2e1 * t1036 * t13 * t3827 + 0.2e1 * t1657 * t840 * r_wheelMntFL_Z + I_body_zz;
t3846 = I_wheel_yy * t995;
t3848 = I_wheel_zz * t995;
t3850 = t7 * r_wheelMntRL_X;
t3852 = t13 * r_wheelMntFR_X;
t3855 = t13 * r_wheelMntRL_X;
t3857 = I_wheel_zz * t1121;
t3861 = t13 * r_wheelMntRR_X;
t3866 = t1036 * t1537 + t3846 * t1946 - t3848 * t1946 - t45 * t3850 + t16 * t3852 + t29 * t3421 + t3 * t3855 - t3857 * t1487 + t2039 * t2921 - t31 * t3453 + t39 * t3861 - t25 * t3162 - t2779 * t2077 - t1168 * t1537;
t3871 = I_wheel_yy * t987;
t3881 = I_wheel_xx * t987;
t3883 = -t2476 * t2921 + t34 * t3852 + t2832 * t2077 + t49 * t3421 + t3871 * t1508 + t51 * t3861 + t10 * t3855 - t18 * t3580 - t1018 * t1517 + t1074 * t1517 - t985 * t1492 + t1014 * t1436 + t1120 * t1492 - t3881 * t1509;
t3884 = t3866 + t3883;
t3885 = t3771 * r_wheelMntFL_X;
t3886 = t3771 * r_wheelMntFR_X;
t3887 = t3771 * r_wheelMntRL_X;
t3888 = t3771 * r_wheelMntRR_X;
t3889 = t3871 * t7;
t3890 = t3846 * t7;
t3891 = I_wheel_yy * t7;
t3892 = t965 * t22;
t3898 = t964 * t22;
t3902 = t870 * t22;
t3904 = t1036 * t139;
t3910 = t29 * t128;
t3914 = t1962 * t139;
t3917 = t1396 * phi_zs1dot;
t3920 = m_wheel * theta_zs1dot;
t3928 = t22 * epsFR_zs1dot;
t3929 = t3928 * t2046;
t3932 = t1120 * t128;
t3934 = t1047 * t128;
t3935 = t1396 * t5;
t3937 = t3892 * r_wheelMntRL_X - t7 * r_airFront_Z * t454 - t1682 * t995 * t7 + t3898 * r_wheelMntRR_X + r_airRear_X * t389 * t7 + t3902 * r_wheelMntFL_X - 0.4e1 * t3904 * t918 * t1825 + t31 * t871 * r_wheelMntFR_X - 0.2e1 * t3910 * t3580 * t993 + 0.2e1 * t2707 * t3914 - 0.2e1 * t2497 * t3917 - 0.2e1 * t3920 * t2743 * zRR_zs - 0.8e1 * t1766 * t3917 + 0.4e1 * t1767 * t3917 + 0.4e1 * t2557 * t3929 + t3932 * t1589 - t3934 * t3935;
t3938 = I_wheel_xx * t128;
t3939 = t2465 * t5;
t3942 = t133 * t1004;
t3945 = I_wheel_zz * t128;
t3946 = t3945 * t1046;
t3948 = t3920 * t7;
t3953 = t3920 * t13;
t3958 = I_wheel_yy * t128;
t3960 = t1037 * t128;
t3962 = t918 * t5;
t3963 = t1040 * t3962;
t3966 = epsRL_zs1dot * psi_zs1dot;
t3967 = t3966 * t13;
t3970 = t152 * t1918;
t3973 = t1055 * psi_zs1dot;
t3976 = t3945 * t993;
t3981 = t1729 * t22;
t3984 = t10 * t128;
t3988 = t3920 * r_wheelMntRR_Y;
t3989 = phi_zs1dot * zRR_zs;
t3993 = t1810 * t5;
t3994 = t1504 * t187;
t3997 = t3548 * t5;
t4000 = t3938 * t3939 - 0.2e1 * t1034 * phi_zs1dot * t3942 + t3946 * t3935 + 0.2e1 * t3948 * zFR_zs1dot * t13 * r_wheelMntFR_Y + 0.2e1 * t3953 * t1033 * t7 * phi_zs1dot - t3958 * t1593 + 0.2e1 * t1036 * t3960 * t3963 + t1435 * t3967 - 0.2e1 * t1439 * t1145 * t3970 + 0.2e1 * t3973 * t3917 + 0.2e1 * t3976 * t1600 - t905 * t119 * zFR_zs + 0.2e1 * t3831 * t3981 - 0.2e1 * t3984 * t1794 * t1370 + 0.4e1 * t3988 * t3989 * t1004 + 0.2e1 * t3993 * t3994 + 0.2e1 * t3958 * t3997;
t4002 = t2748 * epsFR_zs1dot;
t4005 = t1074 * theta_zs1dot;
t4006 = t2432 * t174;
t4014 = t1145 * t174;
t4017 = t1076 * t174;
t4022 = t2168 * t5;
t4024 = t3945 * t1004;
t4032 = t129 * t22;
t4035 = phi_zs1dot * r_wheelMntFR_Z;
t4039 = t1458 * psi_zs1dot;
t4043 = r_wheelMntRL_Y * phi_zs1dot * r_wheelMntRL_Z;
t4046 = -0.2e1 * t1168 * t4002 - 0.2e1 * t4005 * t4006 - 0.2e1 * t2786 * t3942 - 0.2e1 * t1051 * phi_zs1dot * t3942 - 0.2e1 * t3993 * t4014 - 0.2e1 * t3993 * t4017 - t905 * t1165 - t3945 * t3939 + t3945 * t4022 + 0.2e1 * t4024 * t3939 - 0.2e1 * t1802 * t173 * r_wheelMntFR_X - 0.2e1 * t3945 * t3997 - t1051 * t4032 + 0.4e1 * t16 * t1004 * t4035 * t133 + t2907 * t4039 - t905 * t1096 - 0.2e1 * t3920 * t4043;
t4049 = t1014 * t128;
t4050 = t2204 * t5;
t4056 = r_wheelMntFR_Y * psi_zs1dot;
t4060 = t993 * t987;
t4061 = t4060 * t1123;
t4069 = I_wheel_xx * theta_zs1dot;
t4070 = t4069 * t1004;
t4077 = t1051 * t128;
t4083 = t989 * t187;
t4086 = t4069 * t984;
t4087 = t3760 * t2144;
t4091 = t987 * psi_zs1dot;
t4092 = t4091 * t13;
t4094 = -t905 * t181 * r_wheelMntRL_Y + 0.2e1 * t4049 * t4050 - t13 * r_airRear_Y * t394 - t905 * t1202 + 0.2e1 * t123 * t4056 * t22 - 0.2e1 * t3932 * t4061 - t7 * r_airRear_Z * t394 - 0.4e1 * t2747 * t1717 * t2110 - 0.4e1 * t4070 * t1918 - t905 * t119 * zRR_zs + 0.2e1 * t3958 * t4050 + t4077 * t3935 + 0.2e1 * t211 * t1785 * t22 - 0.2e1 * t1120 * t173 * t4083 + 0.2e1 * t4086 * t4087 - t905 * t1322 + t2926 * t4092;
t4097 = t1120 * t152;
t4098 = t1154 * t1937;
t4101 = t985 * t128;
t4103 = t1092 * t128;
t4104 = t4060 * t1927;
t4107 = t4069 * t1013;
t4108 = t1002 * t7;
t4109 = t4108 * t174;
t4112 = t1748 * t139;
t4117 = t1082 * t187;
t4121 = r_DRL * n_gndRL_Y;
t4123 = t929 * t5;
t4125 = t1121 * t128;
t4128 = t1123 * t1154 * t5;
t4141 = t3958 * t993;
t4144 = t1810 * t1154;
t4147 = t870 * t5;
t4149 = t1304 * t7;
t4150 = t4149 * t148;
t4152 = 0.2e1 * t4097 * t4098 - t4101 * t1589 - 0.2e1 * t4103 * t4104 + 0.2e1 * t4107 * t4109 - 0.2e1 * t2627 * t4112 - t905 * t1112 - 0.2e1 * t1036 * t173 * t4117 - t965 * t4 * t4121 + t4123 * t797 + 0.2e1 * t1120 * t4125 * t4128 - 0.2e1 * t123 * r_wheelMntFR_Y * t3942 - 0.2e1 * t10 * t129 * t836 * t1154 - 0.2e1 * t1092 * t173 * t4014 + 0.2e1 * t4141 * t1605 - 0.2e1 * t4144 * t2033 + t4147 * t788 - t2476 * t4150;
t4153 = t1036 * t128;
t4154 = t2604 * t1881;
t4158 = phi_zs1dot * r_wheelMntRR_Z;
t4162 = t741 * t4;
t4163 = r_DFR * n_gndFR_Z;
t4165 = t2204 * t1794;
t4167 = t1427 * psi_zs1dot;
t4169 = t3945 * t998;
t4170 = t3548 * t1794;
t4172 = I_body_zz * t128;
t4180 = I_wheel_zz * theta_zs1dot;
t4185 = t3938 * t993;
t4189 = t1729 * t80;
t4193 = t1729 * t76;
t4202 = -0.2e1 * t4153 * t4154 + 0.4e1 * t39 * t1004 * t4158 * t133 + t4162 * t4163 + t4103 * t4165 - t1851 * t4167 - t4169 * t4170 + t4172 * t3935 + I_wheel_zz * epsRR_zs1dot * t174 + 0.2e1 * t1014 * t173 * t4014 + t2080 * t4167 + 0.2e1 * t4180 * t1002 * t2110 + t3945 * t1593 - 0.2e1 * t4185 * t2664 - 0.2e1 * t29 * t7 * t4189 - 0.2e1 * t10 * t7 * t4193 - 0.2e1 * t1168 * t3960 * t3963 - 0.2e1 * t1784 * t173 * r_wheelMntRL_X;
t4204 = t39 * t128;
t4213 = epsRR_zs1dot * psi_zs1dot;
t4214 = t4213 * t13;
t4216 = t644 * t4;
t4217 = r_DRR * n_gndRR_Z;
t4224 = t1054 * t128;
t4230 = t1724 * t148;
t4234 = t1036 * theta_zs1dot;
t4236 = t1037 * phi_zs1dot * t1039;
t4247 = I_body_yy * t128;
t4249 = -0.2e1 * t4204 * t1794 * t1360 + 0.2e1 * t3953 * t836 * zRL_zs1dot - I_wheel_xx * epsRR_zs1dot * t174 + t1435 * t4214 + t4216 * t4217 - 0.2e1 * t2373 * t3914 - 0.2e1 * t4185 * t1596 + t2864 * t2300 + t4224 * t3935 + 0.4e1 * t10 * t1004 * t3504 * t133 - t3846 * t4230 + 0.2e1 * t4069 * t1918 + 0.2e1 * t4234 * t4236 + 0.4e1 * t3988 * t4158 * t1004 - I_body_xx * t128 * t1896 + 0.2e1 * t123 * t174 * r_wheelMntFR_X - t4247 * t3935;
t4250 = t2107 * t5;
t4257 = I_wheel_yy * theta_zs1dot;
t4264 = t128 * t13;
t4268 = t1927 * t7;
t4271 = t1004 * zFR_zs1dot;
t4275 = t918 * zRR_zs;
t4277 = t3938 * t998;
t4293 = epsRL_zs1dot * t13;
t4294 = t4293 * phi_zs1dot;
t4297 = 0.2e1 * t4250 * t4014 + 0.2e1 * t3948 * phi_zs1dot * t1058 * t13 - 0.2e1 * t4257 * t1002 * t2110 - I_wheel_xx * epsRL_zs1dot * t174 + t4247 * t1896 + t31 * t4264 * r_wheelMntFR_X + 0.2e1 * t1959 * theta_zs1dot * t4268 + 0.2e1 * t3920 * t4271 * r_wheelMntFR_Z - t4216 * t4275 + t4277 * t4170 - 0.2e1 * I_body_yy * theta_zs1dot * t2110 - t1059 * t4032 + 0.2e1 * t3976 * t1596 - t2261 * t2300 + 0.4e1 * t1766 * t2300 + t2351 * t4039 - 0.2e1 * t45 * t129 * t822 * t918 + 0.2e1 * t1047 * t4294;
t4310 = phi_zs1dot * zFR_zs;
t4317 = t1059 * t128;
t4321 = t3938 * t1004;
t4324 = t1729 * t83;
t4330 = t22 * epsFL_zs1dot;
t4331 = t4330 * psi_zs1dot;
t4334 = t388 * t12;
t4339 = -0.2e1 * t1608 * t3967 + 0.2e1 * I_body_zz * theta_zs1dot * t2110 - 0.2e1 * t1128 * t4193 - t905 * t36 - t1691 * t7 - 0.2e1 * t3920 * t4310 * r_wheelMntFR_Y + t3881 * t1121 * t871 * t1013 + t4317 * t3935 - t905 * t27 - t905 * t23 - t4321 * t4022 - 0.2e1 * t39 * t7 * t4324 - t1034 * t4032 + t18 * t871 * r_wheelMntFL_X - 0.2e1 * t1986 * t4331 - t4334 * t2902 * t13 + 0.2e1 * t1635 * t3967;
t4343 = t1014 * t987;
t4344 = t1927 * t148;
t4347 = t1034 * t128;
t4357 = t22 * t1046 * t5;
t4361 = t1729 * t69;
t4371 = t1445 * t187;
t4374 = t128 * t7;
t4375 = t4374 * r_wheelMntRL_X;
t4378 = r_DFR * n_gndFR_X;
t4382 = -t905 * t43 + t3857 * t1668 * t148 - t4343 * t4344 + t3848 * t4230 + t4347 * t3935 - t2584 * t63 + t4334 * t4163 + 0.2e1 * t3881 * t1508 * phi_zs1dot * t984 * t2144 + t3945 * t4357 - 0.2e1 * t3958 * t3935 - 0.2e1 * t1149 * t4361 - 0.2e1 * t25 * t129 * t828 * t918 + 0.2e1 * t211 * t174 * r_wheelMntRL_X + 0.2e1 * t3993 * t4371 + t10 * t4375 - t929 * t12 * t4378 + 0.2e1 * t2873 * t3942;
t4395 = r_DFL * n_gndFL_X;
t4397 = t246 * t12;
t4398 = r_DFL * n_gndFL_Z;
t4400 = t565 * t4;
t4402 = t1154 * r_wheelMntFL_Y;
t4405 = r_DFR * n_gndFR_Y;
t4407 = t985 * t152;
t4412 = m_wheel * t128;
t4425 = t1836 * t1037 * t1039;
t4428 = t3850 * t993;
t4431 = 0.4e1 * t1835 * t1881 * t1154 * phi_zs1dot - 0.4e1 * t3109 * t3929 - t3938 * t4357 + 0.4e1 * t2898 * t4056 * t1154 - t870 * t12 * t4395 + t4397 * t4398 + t4400 * t4398 - t4397 * t4402 - t929 * t4 * t4405 - 0.2e1 * t4407 * t4098 + t45 * t4264 * r_wheelMntRL_X + t4412 * t22 * t1332 * t5 - 0.2e1 * t985 * t3260 * epsFL_zs1dot - 0.2e1 * t2694 * t3917 + 0.2e1 * t985 * t173 * t4083 - 0.4e1 * t4234 * t4425 - 0.2e1 * t3984 * t4428;
t4434 = t985 * theta_zs1dot;
t4436 = t1121 * phi_zs1dot * t988;
t4440 = t1836 * t1121 * t988;
t4445 = t450 * t12;
t4447 = t964 * t5;
t4449 = epsRR_zs1dot * t13;
t4450 = t4449 * phi_zs1dot;
t4457 = r_DRL * n_gndRL_X;
t4461 = t1154 * r_wheelMntRR_Y;
t4463 = t995 * psi_zs1dot;
t4464 = t4463 * t13;
t4466 = t918 * r_wheelMntRR_Z;
t4471 = t1959 * t4167 + t3945 * t1605 - 0.2e1 * t4434 * t4436 - 0.4e1 * t4086 * t4440 + 0.2e1 * t3195 * t4331 + t4445 * t83 + t4447 * t803 - 0.2e1 * t1054 * t4450 + I_wheel_zz * epsRL_zs1dot * t174 - t3958 * t1605 - t965 * t12 * t4457 + 0.2e1 * t1532 * t4112 - t4445 * t4461 + t3651 * t4464 - t4445 * t4466 + 0.2e1 * t2675 * t3917 + t4447 * t801;
t4480 = t4180 * t1004;
t4483 = t1927 * t2163;
t4489 = r_DFL * n_gndFL_Y;
t4491 = t669 * t4;
t4492 = r_DRL * n_gndRL_Z;
t4497 = t387 * t12;
t4499 = t1766 * t5;
t4510 = t1014 * theta_zs1dot;
t4513 = t4216 * t83 + t4447 * t807 - t2619 * t4464 + 0.4e1 * t4434 * t2544 * epsFL_zs1dot + 0.2e1 * t4480 * t2586 - 0.4e1 * t4107 * t4483 - 0.2e1 * t3976 * t1605 - t870 * t4 * t4489 + t4491 * t4492 + 0.2e1 * t1168 * t173 * t4117 + t4497 * t4492 - 0.2e1 * t4499 * t4371 + t4400 * t80 + 0.4e1 * t2647 * t2229 * t1154 - t4216 * t4461 - 0.4e1 * t3948 * t834 * t3504 + 0.4e1 * t4510 * t2110;
t4522 = t4330 * t2046;
t4537 = t1724 * t7;
t4540 = t3920 * t1004;
t4541 = t3729 * r_wheelMntFL_Z;
t4545 = t988 * psi_zs1dot * t2110;
t4558 = t4397 * t80 + 0.2e1 * t3824 * t3981 - 0.2e1 * t49 * t7 * t4189 - 0.2e1 * t4103 * t4050 - 0.4e1 * t3195 * t4522 + 0.2e1 * t3785 * t3981 - 0.2e1 * t3976 * t1593 + 0.2e1 * t1780 * t2842 * t918 - 0.2e1 * t31 * t129 * t830 * t918 - 0.2e1 * t1695 * theta_zs1dot * t4537 + 0.4e1 * t4540 * t4541 + 0.4e1 * t3367 * t4545 - 0.2e1 * t4070 * t2005 + t4147 * t790 - 0.2e1 * t985 * t4125 * t4128 + 0.2e1 * t1022 * t3981 - 0.4e1 * t4257 * t2110;
t4562 = t4180 * t7;
t4564 = t1046 * t13 * phi_zs1dot;
t4574 = t3958 * t1002;
t4579 = t4374 * r_wheelMntFR_X;
t4587 = I_wheel_yy * epsRR_zs1dot;
t4590 = phi_zs1dot * t998 * t996;
t4593 = t2183 * t918;
t4596 = 0.2e1 * t4480 * t2005 + 0.2e1 * t4562 * t4564 + 0.8e1 * t4069 * t2110 + t3938 * t1596 + t4147 * t813 + 0.2e1 * t261 * t174 * r_wheelMntRR_X - t4574 * t3935 + t3476 * t133 - 0.2e1 * t4180 * t2586 + t16 * t4579 - 0.2e1 * t2228 * t173 * r_wheelMntRR_X - t3571 * t4092 - t2456 * t496 + t4123 * t799 - t4587 * t174 - 0.2e1 * t1910 * t4590 + 0.2e1 * t2228 * t4593;
t4597 = t16 * t128;
t4604 = I_wheel_yy * epsRL_zs1dot;
t4607 = t3453 * t993;
t4617 = t3162 * t993;
t4620 = t4412 * t993;
t4623 = t4374 * r_wheelMntRR_X;
t4625 = t867 * r_wheelMntFR_X;
t4634 = -0.2e1 * t4597 * t1794 * t1365 + 0.4e1 * t4434 * t4440 - t2233 * t494 - t4604 * t174 - t2625 * t496 - 0.2e1 * t4597 * t4607 + t4162 * t69 + 0.4e1 * t4510 * t4483 + 0.2e1 * t3920 * t4271 * zFR_zs - t2589 * t494 - 0.2e1 * t4204 * t4617 - 0.2e1 * t4620 * t3053 + t39 * t4623 + t34 * t4625 + t4123 * t805 - t2651 * t494 + 0.2e1 * t1034 * t3981 + 0.2e1 * t2435 * t2300 * t999;
t4645 = t1057 * t128;
t4658 = r_DRR * n_gndRR_X;
t4669 = t1168 * theta_zs1dot;
t4679 = t965 * t5;
t4684 = -0.2e1 * t1022 * phi_zs1dot * t3942 + t4334 * t69 + t25 * t871 * r_wheelMntRR_X - t4645 * t3935 - 0.2e1 * t1851 * theta_zs1dot * t4268 + 0.4e1 * t3264 * t4593 + 0.2e1 * t4250 * t4017 + 0.2e1 * t1784 * t3157 * t918 - t964 * t12 * t4658 + 0.2e1 * t1051 * t3981 + t4412 * t22 * t1139 * t5 - 0.2e1 * t3948 * t1048 * t13 * phi_zs1dot - 0.2e1 * t4669 * t4236 - 0.2e1 * t16 * t129 * t826 * t1154 - 0.2e1 * t211 * r_wheelMntRL_Y * t3942 + t4679 * t809 + t4412 * t22 * t1264 * t5;
t4685 = t2391 * t918;
t4689 = t4069 * t7;
t4690 = t1013 * t13;
t4702 = t1154 * t2144;
t4729 = t867 * r_wheelMntRR_X;
t4731 = 0.4e1 * t3568 * t4685 + t4445 * t4217 - 0.4e1 * t4689 * t4690 * phi_zs1dot - 0.2e1 * t1610 * t4214 - 0.2e1 * t3948 * t1102 * t13 * phi_zs1dot + 0.2e1 * t4086 * t4436 - 0.4e1 * t4097 * t4702 + 0.2e1 * t3920 * t1213 * zRR_zs1dot + 0.2e1 * t3904 * t918 * t2032 - 0.2e1 * t39 * t129 * t832 * t1154 + t4679 * t795 + t4679 * t811 - 0.2e1 * t31 * t13 * t4361 + 0.4e1 * t3728 * t2139 * t133 - 0.2e1 * t3948 * t1108 * t13 * phi_zs1dot + 0.2e1 * t2193 * t3917 + t51 * t4729;
t4748 = t3958 * t996;
t4753 = t2300 * t998;
t4763 = t1074 * t995;
t4764 = t1906 * phi_zs1dot;
t4771 = t1396 * t2304;
t4774 = -0.4e1 * t3953 * t4310 * t799 - 0.2e1 * t4257 * t996 * t2110 + 0.4e1 * t1922 * t3917 + 0.2e1 * t4169 * t3997 + 0.2e1 * t2100 * t4590 - 0.2e1 * t1767 * t1836 * t3548 - t4748 * t3935 + 0.2e1 * t3920 * t3049 * zRL_zs1dot + 0.2e1 * t1810 * t4753 - 0.2e1 * t3364 * t3942 - t1022 * t4032 - 0.2e1 * t18 * t129 * t818 * t918 - 0.2e1 * t4763 * t4764 + t4497 * t76 + 0.2e1 * t1036 * t4002 + t4491 * t76 + 0.2e1 * t2059 * t4771;
t4775 = t31 * t128;
t4788 = t1881 * t148;
t4790 = t1004 * zFL_zs1dot;
t4794 = t3 * t128;
t4803 = t2476 * t139;
t4804 = t918 * t2041;
t4807 = t1187 * t128;
t4809 = t3945 * t996;
t4811 = t1022 * t128;
t4815 = -0.2e1 * t4775 * t3852 * t993 - t3945 * t1600 + t3 * t4375 + 0.2e1 * t4141 * t1593 + 0.2e1 * t2535 * t3942 + 0.2e1 * t4049 * t4104 - t1168 * t995 * t4788 + 0.2e1 * t3920 * t4790 * r_wheelMntFL_Z - 0.2e1 * t4794 * t4428 + t4103 * t1593 + 0.2e1 * t1074 * t173 * t4017 + 0.2e1 * t3823 * t3981 + 0.2e1 * t4803 * t4804 - t4807 * t3935 + t4809 * t3935 + t4811 * t3935 + 0.2e1 * t3776 * t3981;
t4818 = t1018 * theta_zs1dot;
t4819 = t7 * epsFR_zs1dot;
t4820 = t1724 * t4819;
t4824 = r_wheelMntFL_Y * psi_zs1dot;
t4828 = t867 * r_wheelMntRL_X;
t4832 = t1225 * t7;
t4833 = t4832 * t148;
t4835 = t2991 * r_wheelMntRL_Y;
t4841 = t1668 * phi_zs1dot;
t4850 = t3754 * t1825;
t4855 = t1003 * t128;
t4857 = -0.4e1 * t4818 * t4820 + t34 * t4579 + 0.4e1 * t1954 * t4824 * t1154 + t10 * t4828 - 0.2e1 * t2657 * t3917 + t2832 * t4833 + 0.4e1 * t4540 * t4835 - 0.4e1 * t3948 * t820 * t4158 + t1851 * t4841 - 0.2e1 * t4185 * t1600 - 0.2e1 * t4499 * t3994 - 0.2e1 * t1018 * t3981 + t39 * t4729 + 0.2e1 * t4234 * t4850 - t1444 * t3967 + t1092 * t4032 + t4855 * t3935;
t4861 = t133 * t1002;
t4869 = t34 * t128;
t4876 = t25 * t128;
t4893 = t2779 * t139;
t4898 = -0.2e1 * t3945 * t3935 - t1014 * t4032 - 0.2e1 * t3533 * t4861 + 0.4e1 * t3938 * t3935 + t4412 * t22 * t1342 * t5 - 0.2e1 * t4869 * t4607 + 0.2e1 * t1784 * t4685 + t25 * t4264 * r_wheelMntRR_X - 0.2e1 * t4876 * t3861 * t993 - 0.2e1 * t3920 * t4541 - t13 * r_airFront_Y * t454 + 0.2e1 * t2228 * t3126 * t918 + 0.2e1 * t3920 * t1104 * zRL_zs1dot + t51 * t4623 + 0.2e1 * t4818 * t4006 + 0.2e1 * t4893 * t918 * t2781 - t2779 * t4833;
t4906 = phi_zs1dot * zFL_zs;
t4923 = t1030 * t13 * phi_zs1dot;
t4926 = t1103 * t128;
t4933 = t2540 * t918;
t4938 = r_DRR * n_gndRR_Y;
t4946 = -0.2e1 * t1080 * t4294 - 0.2e1 * t3953 * phi_zs1dot * t1010 * t7 - 0.2e1 * t3920 * t4906 * r_wheelMntFL_Y - t1444 * t4214 - 0.2e1 * t1092 * t3981 + 0.2e1 * t4069 * t2586 - 0.2e1 * t3920 * t2743 * r_wheelMntRR_Z - 0.2e1 * t985 * t1145 * t187 * t2144 + 0.2e1 * t4562 * t4923 - t4926 * t3935 - t2080 * t4841 - 0.2e1 * t29 * t129 * t840 * t1154 + 0.4e1 * t2727 * t4933 - t1695 * t4039 - t964 * t4 * t4938 - 0.2e1 * t3953 * phi_zs1dot * t1099 * t7 + 0.4e1 * t4669 * t4425;
t4947 = t867 * r_wheelMntFL_X;
t4952 = I_wheel_zz * phi_zs1dot;
t4955 = t1008 * t128;
t4967 = t1168 * t128;
t4991 = t49 * t4947 - t2700 * t494 - 0.4e1 * t4180 * t2110 + 0.2e1 * t4952 * t4861 - t4955 * t3935 - 0.2e1 * t3009 * t3917 + t45 * t871 * r_wheelMntRL_X - 0.2e1 * t3920 * t4035 * r_wheelMntFR_Y + t3938 * t995 * t1724 * t998 + 0.2e1 * t4967 * t4154 + t1439 * t3967 + 0.2e1 * t3920 * t4790 * zFL_zs + 0.2e1 * t3920 * t1004 * r_wheelMntRR_Z * zRR_zs1dot - 0.2e1 * t3953 * phi_zs1dot * t1186 * t7 + 0.4e1 * t2107 * t3917 - 0.2e1 * t2864 * t3917 + 0.2e1 * t2261 * t3917 - 0.4e1 * t3953 * t4906 * t788;
t5003 = t1011 * t128;
t5005 = t3920 * phi_zs1dot;
t5038 = t29 * t4947 + 0.4e1 * t4005 * t4820 + 0.2e1 * t3948 * phi_zs1dot * t1050 * t13 + t4153 * t1629 - t5003 * t3935 + 0.4e1 * t5005 * zFL_zs * r_wheelMntFL_Y * t1004 + 0.4e1 * t1986 * t4522 - t1959 * t4841 - 0.2e1 * t51 * t7 * t4324 - 0.2e1 * t3910 * t1794 * t1378 - 0.2e1 * t4510 * t4109 - 0.2e1 * t4434 * t4087 - 0.2e1 * t4180 * t2005 - 0.2e1 * t4620 * t1519 * t13 - 0.2e1 * t3 * t7 * t4193 + 0.2e1 * t3948 * zFL_zs1dot * t13 * r_wheelMntFL_Y + 0.2e1 * t2167 * t2300 * t1046;
t5041 = t51 * t128;
t5044 = t1675 * phi_zs1dot;
t5052 = t918 * r_wheelMntFL_Z;
t5058 = t1018 * t995;
t5071 = 0.2e1 * t3766 * t3981 - 0.2e1 * t5041 * t4617 - t2351 * t5044 + 0.2e1 * t3777 * t3981 - 0.2e1 * t4689 * t4923 - t2223 * t494 - t3871 * t4344 - t4397 * t5052 - t4400 * t5052 - t4400 * t4402 - 0.4e1 * t3259 * t4545 + 0.2e1 * t5058 * t4764 + 0.4e1 * t5005 * r_wheelMntFR_Z * r_wheelMntFR_Y * t1004 + 0.2e1 * t1060 * t3981 - t4169 * t1605 + t1036 * t995 * t4788 - t905 * t1857;
t5073 = t1766 * t1154;
t5078 = t187 * t1825;
t5082 = t1123 * t148;
t5085 = t2374 * phi_zs1dot;
t5097 = t4952 * psi_zs1dot;
t5099 = t22 * t1013 * t1002;
t5105 = t3938 * t22;
t5113 = -0.2e1 * t5073 * t3465 + t3 * t4828 - 0.2e1 * t1168 * t1076 * t5078 + t1120 * t987 * t5082 + 0.2e1 * t1092 * t987 * t5085 - t4049 * t4165 - t2907 * t5044 - 0.2e1 * t1184 * t3981 - t905 * t119 * r_wheelMntRR_Z - t905 * t1234 + 0.4e1 * t4540 * t4043 - 0.2e1 * t5097 * t5099 + t3938 * t1600 - t4967 * t1629 + t1439 * t4214 - 0.2e1 * t5105 * t999 * t5 - 0.2e1 * t3953 * phi_zs1dot * t1007 * t7;
t5120 = t4374 * r_wheelMntFL_X;
t5126 = t3928 * psi_zs1dot;
t5140 = I_wheel_xx * phi_zs1dot;
t5141 = t5140 * psi_zs1dot;
t5149 = t1109 * t128;
t5151 = t2039 * t139;
t5154 = t3102 * t918;
t5157 = -t4049 * t1593 - 0.2e1 * t25 * t13 * t4324 - 0.2e1 * t4070 * t2586 + t49 * t5120 - t2474 * t63 - t3945 * t1596 + 0.2e1 * t4101 * t4061 - 0.2e1 * t2557 * t5126 + 0.4e1 * t2390 * t1785 * t1154 + r_airFront_X * t341 * t7 + 0.2e1 * t3953 * t1021 * t7 * phi_zs1dot - 0.2e1 * t1273 * t4189 + 0.2e1 * t5141 * t5099 + 0.2e1 * t3783 * t3981 + 0.2e1 * t159 * t174 * r_wheelMntFL_X - t5149 * t3935 - 0.2e1 * t5151 * t4804 + 0.4e1 * t3027 * t5154;
t5170 = t929 * t22;
t5197 = -0.2e1 * t4689 * t4564 - 0.2e1 * t1003 * t4032 + 0.2e1 * t4049 * t3935 + 0.2e1 * t1802 * t4933 - 0.4e1 * t2435 * t4753 + t5170 * r_wheelMntFR_X - t4763 * t4230 + 0.2e1 * t261 * t2229 * t22 - 0.4e1 * t2059 * t3917 - 0.2e1 * t1059 * phi_zs1dot * t3942 + 0.4e1 * t4407 * t4702 + 0.2e1 * t1653 * t4214 - 0.2e1 * t4277 * t3935 + t1695 * t5044 - 0.4e1 * t4234 * t2470 * epsFR_zs1dot + 0.4e1 * t5005 * zFR_zs * r_wheelMntFR_Y * t1004 - 0.2e1 * t1922 * t4771;
t5232 = -0.2e1 * t4620 * t3659 + 0.2e1 * t1444 * t1145 * t3970 + 0.2e1 * t1055 * t4450 + 0.4e1 * t4562 * t1220 * phi_zs1dot + t2039 * t4150 - 0.4e1 * t4818 * t2110 + 0.4e1 * t4480 * t2124 + t29 * t5120 + 0.2e1 * t4069 * t2005 - t3938 * t4022 + t2908 * t4464 - 0.2e1 * t4343 * t5085 + 0.2e1 * t4180 * t996 * t2110 + 0.2e1 * t1780 * t5154 + 0.4e1 * t1810 * t3917 - 0.2e1 * t1439 * t1076 * t152 * t2124 - t4445 * t4275;
t5254 = t1049 * t128;
t5263 = -t985 * t987 * t5082 + t18 * t4264 * r_wheelMntFL_X + t16 * t4625 + 0.2e1 * t1014 * t3981 + 0.4e1 * t4144 * t2610 - t2548 * t65 - t905 * t1159 - t4334 * t1352 * t7 - 0.2e1 * t4103 * t3935 - 0.2e1 * t261 * r_wheelMntRR_Y * t3942 - t4334 * t1365 * t7 - t5254 * t3935 + t5058 * t4230 - t2578 * t63 - t1679 * t987 * t7 + t2081 * t4092 - 0.2e1 * t3920 * t4835;
t5267 = t5 * t995;
t5309 = t1100 * t128;
t5313 = 0.2e1 * t1036 * t1076 * t5078 + 0.2e1 * t1168 * t5267 * t1834 * t3429 - t1687 * t7 + 0.2e1 * t3953 * t832 * zRR_zs1dot + 0.2e1 * t3109 * t5126 - t4216 * t4466 - 0.2e1 * t1018 * t173 * t4017 - 0.2e1 * t159 * r_wheelMntFL_Y * t3942 + 0.2e1 * t159 * t4824 * t22 + 0.2e1 * t1059 * t3981 + 0.2e1 * t1802 * t2036 * t918 - 0.2e1 * t3948 * t1056 * t13 * phi_zs1dot + 0.2e1 * t2351 * theta_zs1dot * t4537 - 0.2e1 * t34 * t7 * t4361 - 0.2e1 * t1780 * t173 * r_wheelMntFL_X + 0.2e1 * t4169 * t2604 * t1724 - t5309 * t3935 - 0.2e1 * t4669 * t4850;
t5319 = t1047 + t1049 + t1051 + t1022 + I_body_xx - t1053 - t1054 + t1055 + t1057 + t1059 + t1060 + t1063 + t1011 - t1080 + t1100;
t5320 = t1003 + t1101 + t1103 + t1109 + t1008 - t1119 + t1143 + t1034 + t1163 + t1172 - t1184 + t1187 + t1250 + t1253 + t1336 - t1337;
t5326 = I_wheel_zz * t164;
t5327 = t2432 * t13;
t5329 = t4412 * t22;
t5333 = t1396 * theta_zs1dot * t1002;
t5336 = t133 * theta_zs1dot;
t5344 = t2109 * t993;
t5346 = I_wheel_xx * t164;
t5347 = t5346 * t1013;
t5348 = t4108 * t13;
t5350 = t169 * t813;
t5356 = -t905 * t1154 * r_wheelMntFR_Z - 0.2e1 * t4180 * t1873 - t5326 * t5327 + t5329 * t1522 * t181 + 0.2e1 * t1922 * t5333 + 0.2e1 * t1018 * t5336 - t25 * t128 * r_wheelMntRR_Z * t993 + t387 * t5 * t4121 - t4807 * t5344 - t5347 * t5348 - 0.4e1 * t1736 * t5350 - t4574 * t5344 - t905 * t1154 * zFL_zs;
t5357 = t3958 * t22;
t5358 = t1145 * t119;
t5367 = t22 * epsRR_zs1dot * t7;
t5372 = t1076 * t119;
t5374 = t1145 * t139;
t5384 = t152 * t13;
t5385 = t3260 * t5384;
t5388 = t5357 * t5358 - t2418 * t96 + t2098 * t32 - t1312 * t4213 * t7 + t905 * t918 * r_wheelMntFL_Y - t1810 * t5367 + t5329 * t1383 * t181 + t1074 * t191 * t5372 + 0.2e1 * t3267 * t5374 + 0.2e1 * t4876 * r_wheelMntRR_Z * t993 * t1004 + t5329 * t1417 * t181 + t3902 * t818 - 0.4e1 * t3367 * t5385;
t5390 = t4069 * t1145;
t5391 = t7 * t984;
t5408 = t18 * t128;
t5411 = t164 * r_wheelMntFL_Z;
t5419 = t1748 * t13;
t5422 = 0.2e1 * t5390 * t5391 * t2144 + 0.4e1 * t3938 * t5344 - t1092 * t191 * t5358 - t18 * t128 * r_wheelMntFL_Z * t993 - 0.2e1 * t261 * t2183 * t5 - t5329 * t1562 * t119 - t5309 * t5344 + 0.2e1 * t5408 * t3119 - 0.2e1 * t18 * t5411 * t1004 + t1103 * t1998 + t4811 * t5344 - t2356 * t4091 * t7 - 0.2e1 * t4005 * t5419;
t5428 = t1697 * t7;
t5435 = t1082 * t152;
t5448 = t3945 * t22;
t5449 = t1445 * t181;
t5454 = 0.4e1 * t2059 * t2536 - 0.2e1 * t2193 * t2536 - t2625 * t8 + t2352 * t5428 - 0.4e1 * t10 * t139 * t3480 * t169 - t5254 * t5344 - 0.2e1 * t3428 * t5435 - 0.2e1 * t3713 * t2536 - t45 * t128 * zRL_zs * t993 - t31 * t128 * r_wheelMntFR_Z * t993 - 0.2e1 * t1014 * t5336 - t5448 * t5449 - t3003 * t4463 * t7 + t1057 * t1998;
t5458 = t7 * t1030;
t5459 = t5458 * t13;
t5474 = t1071 * t2109;
t5478 = -t4926 * t5344 - t5326 * t5459 - 0.2e1 * t4277 * t5344 + t2578 * t93 - t1696 * t5428 + t1100 * t1998 + t5329 * t1411 * t181 - t2548 * t90 - t29 * t128 * r_wheelMntFL_Y * t993 - 0.2e1 * t3973 * t2536 + t4277 * t5474 - t5149 * t5344 + t1109 * t1998;
t5484 = I_wheel_yy * t164;
t5486 = t1911 * t7;
t5490 = t1445 * t152;
t5494 = t22 * r_DFR * n_gndFR_Z;
t5496 = t3072 * t993;
t5507 = t4172 * t5344 - t1051 * t1998 - 0.2e1 * t39 * t2326 * r_wheelMntRR_Y + t5484 * t5348 + 0.2e1 * t1910 * t5486 + t1049 * t1998 - 0.2e1 * t3267 * t5490 + t2572 * t5494 + 0.2e1 * t4794 * t5496 + t5170 * t12 * r_DFR * n_gndFR_Y - 0.2e1 * t3984 * t822 * t1041 - t4247 * t5344 + t5357 * t5372;
t5516 = t2039 * psi_zs1dot;
t5517 = t1305 * epsRR_zs1dot;
t5520 = t985 * t191;
t5521 = t989 * t181;
t5533 = t25 * t133;
t5537 = theta_zs1dot * r_wheelMntRR_X;
t5541 = -t1022 * t1998 + 0.2e1 * t2476 * t2564 + t5484 * t5327 - 0.2e1 * t123 * t2540 * t5 + 0.2e1 * t5516 * t5517 - t5520 * t5521 + t2584 * t93 - 0.4e1 * t2820 * t228 * t1132 - t2600 * t96 + 0.8e1 * t1766 * t2536 - 0.2e1 * t1120 * phi_zs1dot * t1937 - 0.4e1 * t5533 * t134 * t801 + 0.2e1 * t2116 * t5537 * t801;
t5546 = r_wheelMntFR_Y * t1004 * t993;
t5556 = t1120 * t164;
t5558 = t1004 * t1121 * t988;
t5568 = t49 * psi_zs1dot;
t5576 = -0.2e1 * t3254 * t2536 + t2907 * t2620 + 0.2e1 * t4597 * t5546 - 0.2e1 * t4597 * t799 * t1124 + t1766 * t5367 + t5329 * t1511 * t181 + t4347 * t5344 + 0.2e1 * t5556 * t5558 - 0.2e1 * t5326 * t1387 * t13 - 0.2e1 * t1060 * t5336 + 0.2e1 * t4499 * t2135 - 0.4e1 * t5568 * t228 * t1266 + t5329 * t1380 * t181 - 0.2e1 * t3993 * t2005;
t5583 = t1145 * t1762;
t5591 = t164 * t1121 * t988;
t5599 = t22 * r_DFL * n_gndFL_Z;
t5603 = t1872 * t7;
t5613 = t3898 * t12 * r_DRR * n_gndRR_Y - 0.2e1 * t3614 * t5583 + 0.2e1 * t4818 * t5419 - 0.2e1 * t18 * t2861 + t985 * t5591 - 0.2e1 * t10 * t2878 - 0.4e1 * t1771 * t169 * t797 + t2489 * t5599 - 0.2e1 * t16 * t2327 + 0.2e1 * t1910 * t5603 - t5329 * t1478 * t119 + 0.2e1 * t3984 * t5496 + t3902 * t12 * r_DFL * n_gndFL_Y;
t5617 = t989 * t152;
t5622 = t22 * r_DRL * n_gndRL_Z;
t5631 = t1925 * t7;
t5634 = t164 * t1037 * t1039;
t5640 = -t2671 * t5599 - t2216 * t8 - 0.2e1 * t985 * t293 * t5617 + t2700 * t32 - t2362 * t5622 + t1014 * t191 * t5358 + t2261 * t228 - t39 * t128 * r_wheelMntRR_Y * t993 + t5105 * t5449 + t3487 * t5631 - t1036 * t5634 - t2982 * t87 + 0.2e1 * t850 * t1380 * t152;
t5654 = t128 * t988 * t993;
t5656 = t228 * t1002;
t5661 = t128 * t1004;
t5662 = t5661 * t2688;
t5668 = theta_zs1dot * t1013 * t1002;
t5672 = t2216 * t14 - t5170 * t4 * r_DFR * n_gndFR_X + 0.2e1 * t2694 * t2536 - t5003 * t5344 + 0.2e1 * t1184 * t5336 - 0.2e1 * t25 * t1878 - t1309 * t5654 - 0.2e1 * t1810 * t5656 + 0.2e1 * t4499 * t2005 - 0.2e1 * t1122 * t5662 - 0.2e1 * t2675 * t2536 - 0.2e1 * t2100 * t5668 - t1682 * t1037;
t5675 = t164 * r_wheelMntFR_Z;
t5684 = theta_zs1dot * r_wheelMntFL_X;
t5693 = t164 * r_wheelMntRL_Z;
t5697 = phi_zs1dot * zRL_zs1dot;
t5701 = -0.2e1 * t1789 * t2536 - 0.2e1 * t31 * t5675 * t1004 - t1120 * t5591 - r_airFront_Y * t341 - 0.2e1 * t211 * t3157 * t5 + 0.2e1 * t2116 * t5684 * t813 - t4069 * t4449 + t2719 * t19 + t31 * t164 * zFR_zs - t4069 * t4293 + t45 * t5693 - 0.4e1 * t1766 * t228 + 0.2e1 * t10 * t5697 - r_airRear_Y * t389;
t5704 = t1014 * t164;
t5706 = t1168 * t164;
t5708 = t1004 * t1037 * t1039;
t5711 = t1925 * t2163;
t5715 = t22 * epsRL_zs1dot * t7;
t5717 = t3938 * t1697;
t5720 = t1772 * psi_zs1dot;
t5728 = t1036 * t1723;
t5729 = t1946 * t1825;
t5734 = t5704 * t5348 - 0.2e1 * t5706 * t5708 - 0.2e1 * t1922 * t5711 + t1766 * t5715 - t5717 * t1219 * t1387 - 0.2e1 * t3296 * t5720 + t2589 * t32 + t4855 * t5344 + t4809 * t5344 - t4955 * t5344 - t5448 * t5358 + 0.2e1 * t5728 * t5729 - 0.2e1 * t2261 * t2536;
t5736 = t1036 * t164;
t5759 = t985 * t164;
t5766 = -t5448 * t5372 + 0.2e1 * t5736 * t5708 + t1122 * t5654 - 0.2e1 * t123 * t2036 * t5 + 0.2e1 * t2864 * t2536 - 0.2e1 * t1014 * t1998 + 0.2e1 * t51 * t164 * t803 * t13 - 0.2e1 * t159 * t2842 * t5 - t4169 * t5474 - 0.2e1 * t2381 * t4091 * t4690 + t5346 * t5459 - 0.2e1 * t5759 * t5558 - 0.2e1 * t4204 * t828 * t1041 + t1168 * t5634;
t5770 = t985 * t1915;
t5780 = t5661 * t1837;
t5800 = -0.2e1 * t3945 * t5344 - 0.2e1 * t5770 * t1508 * t2144 + t905 * t918 * r_wheelMntRR_Y - t2244 * t8 + 0.2e1 * t5346 * t3311 * t13 - 0.2e1 * t1038 * t5780 + 0.2e1 * t4069 * t1873 + 0.2e1 * t4204 * t1004 * r_wheelMntRR_Y * t993 - t905 * t1154 * zRL_zs + 0.2e1 * t850 * t1519 * t139 - t3304 * t5494 - t905 * t1154 * r_wheelMntRR_Z + 0.2e1 * t4952 * t997 * t2032;
t5817 = theta_zs1dot * t998 * t996;
t5829 = 0.2e1 * t3484 * t2536 - 0.4e1 * t1810 * t2536 - 0.2e1 * t1059 * t5336 + 0.2e1 * t49 * t164 * t790 * t13 - t5326 * t5348 + t4224 * t5344 - t3 * t128 * r_wheelMntRL_Y * t993 + 0.2e1 * t1910 * t5817 + 0.2e1 * t261 * t4158 - t3902 * t840 + t25 * t1877 + t1011 * t1998 - 0.2e1 * t1022 * t5336 - 0.2e1 * t2167 * t2347;
t5839 = t1697 * t4819;
t5847 = t128 * t1039 * t993;
t5858 = t1435 * theta_zs1dot;
t5859 = t1076 * t139;
t5862 = 0.2e1 * t1092 * t5336 - 0.2e1 * t3993 * t2135 - t4748 * t5344 + 0.2e1 * t1722 * t5839 + t2625 * t14 + 0.2e1 * t1309 * t5662 + t2660 * t93 - t1169 * t5847 + t5170 * t824 + 0.2e1 * t3910 * r_wheelMntFL_Y * t1004 * t993 - 0.2e1 * t2100 * t5603 + 0.2e1 * t3171 * t2536 - 0.2e1 * t5858 * t5859;
t5870 = t7 * t1046;
t5871 = t5870 * t13;
t5874 = t1082 * t181;
t5886 = t1504 * t152;
t5892 = 0.2e1 * t3 * t164 * t809 * t13 + t3898 * t820 + t2474 * t93 - t2548 * t96 + t5346 * t5871 + t1036 * t191 * t5874 + 0.2e1 * t4069 * t3610 + t3946 * t5344 - 0.2e1 * t211 * t2391 * t5 - t2180 * t87 - 0.2e1 * t159 * t3102 * t5 + 0.2e1 * t1871 * t5886 - t16 * t128 * r_wheelMntFR_Y * t993;
t5921 = -0.4e1 * t3056 * t134 * t799 + t1008 * t1998 - 0.4e1 * t1471 * t1772 * t2391 + 0.2e1 * t2122 * t4463 * t1220 - t3938 * t7 * t1031 * t13 + 0.4e1 * t2747 * t2748 * t5384 + t4077 * t5344 - t4645 * t5344 + t1038 * t5847 + 0.2e1 * t2116 * t5684 * t788 - 0.2e1 * t1051 * t5336 + 0.2e1 * t2657 * t2536 + t25 * t3211;
t5923 = t1076 * t2915;
t5927 = t1504 * t181;
t5946 = t1851 * t2082 - 0.2e1 * t2481 * t5923 + t2244 * t14 + t5105 * t5927 - t5448 * t5927 + 0.2e1 * t1871 * t5490 + 0.2e1 * t850 * t1511 * t152 + t2223 * t19 - t2692 * t90 + t2719 * t32 - 0.2e1 * t1034 * t5336 - 0.4e1 * t3387 * t228 * t1213 - t1810 * t5715 - t669 * t5 * t4457;
t5963 = t1015 * t2109;
t5975 = 0.2e1 * t1767 * t1396 * t3700 - t3576 * t228 - 0.4e1 * t2107 * t2536 - 0.2e1 * t4103 * t5344 - 0.2e1 * t1810 * t2838 - t2962 * t5631 - t905 * t1154 * r_wheelMntFL_Z - t1034 * t1998 + t4103 * t5963 + 0.2e1 * t2116 * t5537 * t803 - t2600 * t90 + 0.2e1 * t985 * phi_zs1dot * t1937 - 0.2e1 * t3910 * t818 * t1041;
t5982 = theta_zs1dot * r_wheelMntFR_X;
t6002 = -0.2e1 * t2435 * t3517 - t2660 * t87 + 0.2e1 * t1916 * t1893 * t4690 + 0.2e1 * t2116 * t5982 * t797 + 0.2e1 * t3009 * t2536 - t2456 * t8 + t2223 * t32 + t18 * t2860 + t2700 * t19 - t3902 * t4 * r_DFL * n_gndFL_X + 0.2e1 * t2458 * t2536 + t5329 * t1497 * t181 - t5329 * t1453 * t119 + t2098 * t19;
t6018 = t1168 * t191;
t6026 = -t2153 * t87 - 0.2e1 * t2808 * t2536 - 0.2e1 * t1767 * t5839 + t2233 * t32 - 0.2e1 * t2059 * t5333 + 0.2e1 * t2116 * t5982 * t805 + 0.2e1 * t159 * t2139 - t2864 * t228 - t6018 * t5874 + t905 * t918 * r_wheelMntRL_Y + t4180 * t4293 - t644 * t5 * t4658 + t2589 * t19;
t6027 = t1018 * t164;
t6041 = t22 * r_DRR * n_gndRR_Z;
t6058 = -t6027 * t5327 + 0.2e1 * t261 * t3989 - 0.2e1 * t2500 * t2536 + t45 * t164 * zRL_zs - 0.2e1 * t45 * t5693 * t1004 + 0.2e1 * t159 * t4906 + t2848 * t6041 + t450 * t5 * t4938 + 0.2e1 * t3945 * t7 * t1025 * t13 - t2584 * t87 - 0.2e1 * t261 * t3126 * t5 + t4317 * t5344 + 0.2e1 * t5326 * t2109 - 0.2e1 * t3267 * t5886;
t6084 = -I_body_zz * t164 * t2109 - t1312 * t3966 * t7 - t1679 * t1121 + I_body_yy * t164 * t2109 - t905 * t1154 * zRR_zs - 0.2e1 * t4180 * t3610 + 0.2e1 * t2116 * t5982 * t799 + t5329 * t1539 * t181 + t2153 * t93 + 0.2e1 * t5484 * t2109 - t3892 * t836 + t3892 * t834 - t2474 * t87;
t6107 = -t2692 * t96 - 0.2e1 * t5140 * t997 * t2032 + t3902 * t838 - t3898 * t832 - t4049 * t5963 + t2371 * t32 - t2578 * t87 + t3892 * t822 - 0.2e1 * t5858 * t5374 + 0.2e1 * t1169 * t5780 - 0.4e1 * t1835 * t1881 * t2506 + 0.2e1 * t1036 * t293 * t5435 - 0.2e1 * t2768 * t5517;
t6120 = t1962 * t13;
t6137 = 0.2e1 * t2943 * t5923 + t2456 * t14 + 0.2e1 * t2107 * t5656 + t2233 * t19 - t3892 * t4 * r_DRL * n_gndRL_X + 0.4e1 * t2435 * t2838 + 0.2e1 * t4107 * t6120 - t905 * t1154 * zFR_zs + 0.2e1 * t1120 * t293 * t5617 + 0.4e1 * t3259 * t5385 + 0.2e1 * t1018 * t1998 - 0.4e1 * t5533 * t134 * t803 - t5329 * t1519 * t119;
t6142 = t1168 * t1723;
t6155 = t1074 * t164;
t6160 = -t1829 * t87 - 0.4e1 * t5346 * t2109 - t2351 * t2620 - 0.2e1 * t6142 * t5729 + t4180 * t4449 + t2371 * t19 + t31 * t5675 - 0.2e1 * t4510 * t6120 - t5326 * t5871 + t2089 * t5622 - 0.2e1 * t5140 * t2005 + t1829 * t93 + t6155 * t5327 + t3892 * t12 * r_DRL * n_gndRL_Y;
t6186 = t2982 * t93 + 0.2e1 * t123 * t4035 - 0.4e1 * t45 * t152 * t1370 * t134 + 0.2e1 * t1910 * t5668 + 0.2e1 * t2779 * phi_zs1dot * t1225 * epsRL_zs1dot - t2418 * t90 + t18 * t5411 - t3934 * t5344 - 0.2e1 * t3958 * t5344 + t2651 * t32 + t905 * t918 * r_wheelMntFR_Y + t4587 * t134 + t4604 * t134;
t6190 = t1120 * t191;
t6211 = -0.4e1 * t49 * t133 * t5350 + t6190 * t5521 - 0.4e1 * t1922 * t2536 + 0.2e1 * t2553 * t5583 - t905 * t1154 * r_wheelMntRL_Z - 0.2e1 * t3993 * t2209 - t5170 * t826 + t5170 * t830 + t3898 * t828 - t1059 * t1998 - 0.2e1 * t2201 * t2536 - 0.2e1 * t5140 * t2586 + t2180 * t93 + 0.2e1 * t3 * t5697;
t6239 = 0.2e1 * t123 * t4310 + t2651 * t19 - t741 * t5 * t4378 + 0.2e1 * t4049 * t5344 + t388 * t5 * t4405 - 0.4e1 * t1767 * t2536 - t565 * t5 * t4395 + t2080 * t2082 - 0.2e1 * t2100 * t5817 - 0.2e1 * t2100 * t5486 + 0.2e1 * t4499 * t2209 + 0.2e1 * t2116 * t5537 * t807 + 0.2e1 * t2116 * t5684 * t790;
t6267 = 0.2e1 * t2059 * t5711 + t246 * t5 * t4489 + t1695 * t2620 + 0.2e1 * t2497 * t2536 - 0.2e1 * t3683 * t5720 + 0.2e1 * t3267 * t5859 + 0.2e1 * t2815 * t5720 - 0.2e1 * t1074 * t293 * t5859 + 0.2e1 * t34 * t164 * t1551 + 0.2e1 * t4869 * t5546 + t1187 * t1998 - t3898 * t4 * r_DRR * n_gndRR_X - t2636 * t6041 - t1959 * t2082;
t6277 = F_DSFL;
t6278 = t5661 * t993;
t6280 = t228 * t2109;
t6291 = t2671 * t13 - t2489 * t13 - t3910 - t49 * t128 - t4400 * t119 + t6277 + t29 * t6278 - 0.2e1 * t3579 * t6280 + t5408 * t5344 - t5329 * t80 * t7 + 0.2e1 * t3420 * t2536 + 0.2e1 * t2116 * t5684 * t13;
t6294 = t173 * phi_zs1dot;
t6301 = t792 * t7 * g;
t6311 = -0.2e1 * t5568 * t6280 + 0.2e1 * t49 * t6294 - t18 * t1998 - 0.2e1 * t18 * t5336 + t6301 - t29 * t2326 - t49 * t2326 - t4397 * t119 + 0.2e1 * t29 * t6294 + t49 * t6278 - t29 * t148 - t918 * t870 - t49 * t148;
t6328 = 0.2e1 * t34 * t6294 + 0.2e1 * t16 * t6294 - t4597 - t4869 - t16 * t148 - t2572 * t13 + t3304 * t13 - t918 * t929 + t4775 * t5344 - t31 * t1998 - 0.2e1 * t31 * t5336 + 0.2e1 * t2116 * t5982 * t13;
t6340 = F_DSFR;
t6347 = -t5329 * t69 * t7 - 0.2e1 * t2820 * t6280 + t6301 - 0.2e1 * t34 * psi_zs1dot * t6280 + 0.2e1 * t31 * psi_zs1dot * t2536 + t16 * t6278 + t6340 - t16 * t2326 - t34 * t2326 - t4334 * t119 - t4162 * t119 - t34 * t148 + t34 * t6278;
t6365 = -t10 * t148 - t3 * t148 - t4794 - t918 * t965 + t2362 * t13 - t2089 * t13 - t5329 * t76 * t7 - 0.2e1 * t3071 * t6280 - 0.2e1 * t2066 * t6280 + 0.2e1 * t2881 * t2536 + 0.2e1 * t2116 * t2882 + t10 * t6278;
t6366 = F_DSRL;
t6381 = t6366 + t3 * t6278 + 0.2e1 * t10 * t6294 - 0.2e1 * t45 * t5336 - t45 * t1998 + 0.2e1 * t3 * t6294 + t6301 - t4497 * t119 - t3 * t2326 - t4491 * t119 - t10 * t2326 + t45 * t128 * t5344 - t3984;
t6396 = t2636 * t13 - t2848 * t13 - t918 * t964 - t5041 - t4204 - t39 * t148 - t51 * t148 - t5329 * t83 * t7 + 0.2e1 * t2116 * t5537 * t13 + t51 * t6278 + t39 * t6278 - t25 * t1998;
t6411 = F_DSRR;
t6416 = 0.2e1 * t39 * t6294 + 0.2e1 * t51 * t6294 - 0.2e1 * t25 * t5336 + 0.2e1 * t25 * psi_zs1dot * t2536 - 0.2e1 * t2742 * t6280 + t6301 - 0.2e1 * t3387 * t6280 + t4876 * t5344 + t6411 - t51 * t2326 - t4445 * t119 - t4216 * t119 - t39 * t2326;
t6420 = r_DFL * t870;
t6421 = t6420 * t987;
t6425 = t1145 * t174 * t988;
t6429 = t1145 * t181 * t988;
t6435 = t1005 * t988;
t6442 = t228 * t1761;
t6445 = t1015 * t988;
t6451 = t3745 * t4;
t6452 = t1427 * n_gndFL_Z;
t6456 = t228 * t2046;
t6464 = t5 * t984 * t1936;
t6467 = t1915 * t139;
t6472 = -0.2e1 * t3932 * t6445 + t6451 * t6452 - t5858 * t4092 + t1313 * t153 - 0.4e1 * t1986 * t6456 + t3267 * t4092 - t1670 * t5336 - t3078 * t1314 * n_gndFL_X + 0.2e1 * t5097 * t6464 - 0.2e1 * t2707 * t6467 + 0.2e1 * t5347 * t4268;
t6478 = t5391 * t988;
t6484 = t1260 * t7;
t6489 = t3760 * t988;
t6492 = t228 * t2772 * t988;
t6498 = t3078 * t12;
t6500 = t1015 * t2544;
t6504 = t6420 * t5;
t6509 = t6420 * t22;
t6520 = t148 * t1002 * t988;
t6526 = t181 * t987 * n_gndFL_Z;
t6528 = -t6498 * t6452 - t4101 * t6500 + 0.2e1 * t6190 * t6429 + t6504 * t987 * t12 * t13 * n_gndFL_Y - t6509 * t1121 * t4 * n_gndFL_X + t6509 * t1121 * t12 * n_gndFL_Y + t3078 * t22 * t1668 * n_gndFL_X - t985 * t6520 - 0.2e1 * t5141 * t6464 - t3871 * t3089 + t6451 * t6526;
t6556 = I_wheel_xx * t1121;
t6568 = -t3857 * t128 * t5344 - t4180 * t4841 + t1120 * t6520 + t3932 * t6500 - t6556 * t5336 - t2100 * t1853 - t985 * t5654 + 0.2e1 * t6556 * t22 * t5720 + 0.2e1 * t4101 * t6435 - t5556 * t6489 - 0.2e1 * t1259 * t5720;
t6576 = t128 * t1002 * t988;
t6584 = t1487 * n_gndFL_Z;
t6587 = t4374 * t1124;
t6595 = 0.2e1 * t2373 * t6467 - 0.2e1 * t2553 * t6425 + t1120 * t5654 + t1120 * t6576 + t3745 * t1314 * n_gndFL_Y - 0.2e1 * t985 * t2326 * t988 + t3745 * t12 * t6584 - t5346 * t4268 + 0.2e1 * t3195 * t6587 + t1910 * t1853 + 0.2e1 * t5346 * t1004 * t984 * t988;
t6609 = t1925 * t187;
t6616 = -t985 * t6576 + 0.2e1 * t1916 * t1893 * t6478 - t1679 - t1871 * t4092 + t3078 * t4 * t6584 - 0.2e1 * t3195 * t5336 + 0.4e1 * t3195 * t6456 + t6556 * t128 * t5344 + 0.2e1 * t1922 * t6609 - 0.2e1 * t2059 * t6609 - 0.2e1 * t1986 * t6587;
t6624 = t1712 * t4;
t6626 = t181 * t995 * n_gndFR_Z;
t6635 = t3754 * t1039;
t6637 = t1710 * t12;
t6638 = t1458 * n_gndFR_Z;
t6648 = t2436 * t1039;
t6653 = I_wheel_zz * t1037;
t6662 = r_DFR * t929;
t6663 = t6662 * t22;
t6667 = t2134 * t1039;
t6670 = -0.2e1 * t3904 * t228 * t2432 * t1039 + 0.2e1 * t3109 * t6587 + 0.2e1 * t4024 * t6648 + t6624 * t6638 - t4180 * t5044 + t6653 * t5336 - 0.2e1 * t6653 * psi_zs1dot * t2536 + t1710 * t22 * t1675 * n_gndFR_X + t1910 * t3004 + t6663 * t1037 * t12 * n_gndFR_Y - 0.2e1 * t4185 * t6667;
t6672 = t5267 * t7;
t6677 = t6662 * t5;
t6694 = I_wheel_xx * t1037;
t6699 = t6662 * t995;
t6702 = I_wheel_xx * t148;
t6705 = t1076 * t174 * t1039;
t6710 = t1946 * t2239;
t6715 = t164 * t1039;
t6726 = -I_wheel_zz * t148 * t6667 - t6699 * t87 * n_gndFR_Y + t6702 * t6667 + 0.2e1 * t2481 * t6705 + 0.2e1 * t4005 * t5044 - 0.2e1 * t5728 * t6710 + 0.2e1 * t4169 * t1698 + t1168 * t6715 - t1036 * t6715 - 0.2e1 * t4153 * t1005 * t1039 + 0.2e1 * t5717 * t1219 * t13 * t997 * t1039;
t6730 = phi_zs1dot * t997 * t2031;
t6738 = t1071 * t2470;
t6743 = t1697 * t187;
t6764 = t1723 * t139;
t6772 = -0.2e1 * t1722 * t6743 + t6694 * t128 * t5344 - t1871 * t4464 + 0.2e1 * t4144 * t169 * t6667 - 0.4e1 * t2557 * t6456 + 0.2e1 * t4967 * t1071 * t1039 - 0.2e1 * t6155 * t4537 + 0.2e1 * t2627 * t6764 - 0.4e1 * t4144 * t169 * t2123 - t5736 * t6635 - t5858 * t4464;
t6794 = t1318 * t153 + 0.4e1 * t3904 * t228 * t1881 - t3846 * t3089 - t2100 * t3004 - t6663 * t1037 * t4 * n_gndFR_X - 0.2e1 * t2943 * t6705 - 0.2e1 * t4818 * t5044 + t3267 * t4464 - t6637 * t6626 - 0.2e1 * t4499 * t6730 + 0.2e1 * t6694 * t22 * t5720;
t6796 = t1441 * n_gndFR_Z;
t6823 = t1710 * t4 * t6796 - 0.2e1 * t1532 * t6764 - t6699 * t19 * n_gndFR_X + t5105 * t6672 - 0.2e1 * t3428 * t1076 * t152 * t1039 + 0.2e1 * t2557 * t5336 - t1682 + t1712 * t12 * t6796 - t6677 * t995 * t4 * t13 * n_gndFR_X - 0.2e1 * t6018 * t1076 * t181 * t1039 + 0.2e1 * t2122 * t4463 * t2030 * t1039;
t6828 = theta_zs1dot * psi_zs1dot * t13;
t6829 = t1439 * t6828;
t6830 = t3945 * t3962;
t6831 = t918 * phi_zs1dot;
t6832 = t1810 * t6831;
t6833 = r_DRL * t965;
t6836 = t6833 * t5;
t6849 = t4180 * t174;
t6850 = -t6829 - t6830 + t6832 - t6833 * t19 * n_gndRL_X + t6836 * t14 * n_gndRL_Y - t6836 * t90 * n_gndRL_X + t3743 * t87 * n_gndRL_Z - t1685 * t1154 * n_gndRL_Y + t3743 * t1154 * n_gndRL_X - 0.2e1 * t4069 * t4564 - t6849;
t6852 = t1435 * t6828;
t6853 = t2441 * t7;
t6856 = t1312 * t153;
t6864 = t4257 * t174;
t6865 = t4069 * t174;
t6866 = t1444 * t6828;
t6867 = -t3945 * t1504 - t6852 + 0.2e1 * t5448 * t6853 + t6856 + t6702 * t1504 - t2779 * t148 * t1225 + t5326 * t1504 + t2832 * t128 * t1225 - t5346 * t1504 - t6864 + t6865 + t6866;
t6869 = t3938 * t3962;
t6872 = t5870 * phi_zs1dot;
t6876 = t1004 * t1045 * t1225;
t6878 = t1766 * t6831;
t6880 = t993 * t1045 * t1225;
t6885 = t1005 * t1225;
t6889 = t6869 + t1685 * t19 * n_gndRL_Z - 0.2e1 * t1910 * t6872 + t5346 * t6876 - t6878 - t3938 * t6880 - t5326 * t6876 + t3945 * t6880 - t1687 - t2832 * t128 * t6885 + t3945 * t1045 * t6885;
t6894 = phi_zs1dot * t1045 * t1225;
t6898 = t181 * n_gndRL_Z;
t6911 = t1046 * psi_zs1dot * t13;
t6920 = -0.2e1 * t4893 * t228 * t4832 + 0.2e1 * t3993 * t6894 + t1685 * t4 * t6898 - t6833 * t87 * n_gndRL_Y + 0.2e1 * t5073 * t2682 + 0.2e1 * t4180 * t4564 - 0.2e1 * t4499 * t6894 + 0.2e1 * t2100 * t6872 + 0.2e1 * t1871 * t6911 - t3743 * t12 * t6898 - 0.2e1 * t5105 * t6853 - 0.2e1 * t3267 * t6911;
t6924 = t1030 * psi_zs1dot * t13;
t6927 = t2197 * t1304;
t6929 = r_DRR * t964;
t6930 = t6929 * t5;
t6933 = -t6829 - t6830 + t6832 + 0.2e1 * t1871 * t6924 - t6849 - t3938 * t6927 - t6852 + t6930 * t14 * n_gndRR_Y + t6856 - t6864 + t6865;
t6947 = t6866 + t6869 + t6702 * t1445 - t5346 * t1445 - t2476 * t148 * t1304 - t2476 * t128 * t1304 - t6878 - t1691 + t3938 * t1445 + t3552 * t19 * n_gndRR_Z - t6929 * t19 * n_gndRR_X - t6930 * t90 * n_gndRR_X;
t6956 = t181 * n_gndRR_Z;
t6964 = t5 * phi_zs1dot * t1304;
t6970 = t228 * t4149;
t6973 = t3145 * t7;
t6976 = t3591 * t1154 * n_gndRR_X - t6929 * t87 * n_gndRR_Y + t3591 * t87 * n_gndRR_Z + t3552 * t4 * t6956 - t3552 * t1154 * n_gndRR_Y - t3591 * t12 * t6956 + t3945 * t6927 + 0.2e1 * t2768 * t6964 + t2476 * t128 * t1005 * t1304 - 0.2e1 * t4803 * t6970 + 0.2e1 * t5448 * t6973;
t6981 = t1004 * t1029 * t1304;
t6990 = t5458 * phi_zs1dot;
t7000 = t5326 * t1445 + 0.2e1 * t5151 * t6970 - t5326 * t6981 - 0.2e1 * t5105 * t6973 - 0.2e1 * t3267 * t6924 + 0.2e1 * t4180 * t4923 - t4321 * t6927 - 0.2e1 * t1910 * t6990 - 0.2e1 * t4069 * t4923 - 0.2e1 * t5516 * t6964 + t5346 * t6981 + 0.2e1 * t2100 * t6990;
gg(1,1) = t2;
gg(1,4) = t61;
gg(1,5) = t86;
gg(1,6) = t118;
gg(1,7) = t122;
gg(1,8) = t122;
gg(1,9) = t122;
gg(1,10) = t122;
gg(1,15) = (t194 + t237 + t282 + t323 + t360 + t392 + t427 + t456);
gg(2,2) = t2;
gg(2,4) = t490;
gg(2,5) = t510;
gg(2,6) = t537;
gg(2,7) = t540;
gg(2,8) = t540;
gg(2,9) = t540;
gg(2,10) = t540;
gg(2,15) = (t567 + t598 + t637 + t664 + t697 + t723 + t754 + t783);
gg(3,3) = t2;
gg(3,5) = t817;
gg(3,6) = t842;
gg(3,7) = t843;
gg(3,8) = t843;
gg(3,9) = t843;
gg(3,10) = t843;
gg(3,15) = (t881 + t915 + t946 + t981);
gg(4,1) = t61;
gg(4,2) = t490;
gg(4,4) = (t1052 + t1090 + t1137 + t1177 + t1208 + t1251 + t1299 + t1346);
gg(4,5) = t1573;
gg(4,6) = t1656;
gg(4,7) = t1660;
gg(4,8) = t1663;
gg(4,9) = t1665;
gg(4,10) = t1667;
gg(4,11) = t1672;
gg(4,12) = t1677;
gg(4,13) = t1678;
gg(4,14) = t1678;
gg(4,15) = (-0.4e1 * t1120 * t1759 * t1763 - 0.2e1 * t985 * t1925 * t1930 + 0.4e1 * t1766 * t2604 * t2121 * t1220 - t1682 * t22 * t1675 + t1679 * t5 * t1121 + 0.2e1 * t1780 * t1350 * t169 + 0.4e1 * t985 * t1894 * t1898 + 0.4e1 * t1771 * t1772 * t1158 - 0.4e1 * t2435 * t2465 * t293 - 0.2e1 * t1702 * t1453 * t13 - 0.4e1 * t1014 * t2016 * t2018 - 0.4e1 * t2182 * t2183 * t1005 + t1682 * t5 * t1037 - t1851 * t22 * t1853 - 0.2e1 * t1784 * t1785 * t1041 + t1081 * t1744 + 0.4e1 * t1702 * t1453 * t1124 + 0.2e1 * t2143 * t1937 - 0.2e1 * t1051 * t22 * t1816 + 0.4e1 * t1168 * t1946 * t1407 * t3089 + 0.2e1 * t2535 * t3085 + 0.4e1 * t985 * t1759 * t1763 - t1679 * t22 * t1668 - 0.2e1 * t39 * t173 * t1865 + t3078 * n_gndFL_X - 0.2e1 * t1702 * t1562 * t13 - 0.2e1 * t2107 * t1697 * t2287 + 0.4e1 * t2390 * t2391 * t1124 + 0.2e1 * t1036 * t1697 * t2241 + t3414 + 0.2e1 * t2228 * t1358 * t169 + 0.2e1 * t2167 * t2197 * t2041 + 0.2e1 * t3034 * t2540 * t993 + 0.2e1 * t1810 * t1888 * t1890 + 0.4e1 * t1702 * t1522 * t1041 - t18 * t7 * t2717 - 0.4e1 * t1074 * t2016 * t1725 + t3 * t13 * t2711 + 0.2e1 * t2321 * t2155 + 0.4e1 * t1855 * t1772 * t1578 + 0.4e1 * t2898 * t2902 * t134 + 0.4e1 * t2898 * t2540 * t1124 + t29 * t13 * t2717 + t1080 * t13 * t232 + 0.2e1 * t2841 * t2842 * t993 - 0.2e1 * t1766 * t2957 * t2959 - 0.2e1 * t1120 * t2678 * t2145 - 0.4e1 * t2012 * t1755 * zRR_zs + 0.2e1 * t1153 * t3211 * t1004 - 0.4e1 * t985 * t1893 * t2545 - t1325 * t2324 + 0.4e1 * t3420 * t3161 * t3421 + 0.2e1 * t2476 * t1154 * t2042 + 0.4e1 * t1771 * t169 * t1112 + t1831 - 0.2e1 * t1702 * t1383 * t7 + 0.2e1 * t1008 * t22 * t1816 + t3244 + t3124 + 0.2e1 * t1109 * t7 * t1730 - 0.4e1 * t1722 * t3548 * t293 + 0.4e1 * t1464 * t1755 * t3118 - 0.4e1 * t985 * t2016 * t2517 + 0.4e1 * t2397 * t2150 - 0.2e1 * t2476 * t5 * t2564 + t10 * t13 * t2711 + 0.2e1 * t3428 * t1076 * t3429 - 0.4e1 * t3647 * t169 * t1825 + t2153 * t8 - t1695 * t2344 + 0.2e1 * t3117 * t119 * t27 + 0.2e1 * t1057 * t22 * t1816 - 0.2e1 * t2497 * t1768 + t1217 * t1820 - 0.4e1 * t1835 * t1838 + 0.2e1 * t1277 * t2327 - 0.2e1 * t1038 * t2471 - t2908 * t2620 + t1933 - 0.2e1 * t1841 * t1596 + t3306 - 0.2e1 * t2039 * t1154 * t2042 + t2670 - 0.2e1 * t1049 * t1861 - t2660 * t14 + t2008 + 0.4e1 * t1367 * t232 + t2474 * t8 + 0.4e1 * t2012 * t1755 * t1213 + 0.2e1 * t1789 * t1768 + t2584 * t8 + 0.2e1 * t3254 * t1795 - 0.2e1 * t51 * t173 * t1865 + 0.2e1 * t2707 * t2375 + t2514 + t3001 + t3642 - t25 * t7 * t1849 - t1651 * t1998 + 0.2e1 * t1258 * t2856 - 0.2e1 * t1217 * t1046 * t2023 + 0.2e1 * t2193 * t1768 - 0.2e1 * t2133 * t2209 + t2692 * t32 + 0.4e1 * t1855 * t1858 - 0.4e1 * t2837 * t2838 + 0.2e1 * t1789 * t1795 - t2113 * t1505 - 0.2e1 * t1100 * t1861 - 0.2e1 * t2335 * t1861 + t3651 * t2620 + t1959 * t2428 - t1971 * t3312 - t1969 * t1381 + 0.2e1 * t2888 * t1795 + 0.2e1 * t2201 * t1795 - t1303 * t2922 + t3613 + 0.4e1 * t1168 * t2172 * t2174 + t3472 + t2418 * t32 + t3720 + t2702 - 0.8e1 * t2251 * t2893 + t2848 * t23 + t3187 - 0.2e1 * t1871 * t1873 + 0.2e1 * t1802 * t2596 - t1258 * t1820 - 0.2e1 * t2029 * t2033 + t3694 + t1969 * t1520 - t2244 * t93 - 0.4e1 * t1935 * t2853 + t3497 + t1746 + t2281 + t2891 + t3362 + 0.2e1 * t3109 * t3247 + 0.2e1 * t31 * t173 * t187 * t36 - 0.2e1 * t1217 * t2856 - 0.2e1 * t2341 * t1861 + t2246 - 0.2e1 * t1481 * t232 + t2641 + 0.2e1 * t123 * t2036 + t3529 + t2091 - 0.2e1 * t1766 * t2586 + t3279 - t2719 * t90 + 0.2e1 * t3066 * t1861 + t3062 - 0.2e1 * t2100 * t2486 - t1435 * t1976 - t2474 * t14 + 0.4e1 * t1767 * t1768 + t2600 * t32 - 0.8e1 * t2167 * t1897 + t1230 * t3069 - 0.2e1 * t3171 * t1795 - 0.2e1 * t1008 * t1861 + t2550 + t986 * t2271 - 0.4e1 * t2059 * t2205 + t1439 * t1993 + t1973 + 0.2e1 * t2100 * t2442 + t3160 + t3031 + t3586 + t2132 + 0.4e1 * t2727 * t2596 + 0.4e1 * t2100 * t1912 + 0.2e1 * t1532 * t2628 - 0.2e1 * t2261 * t1897 - 0.2e1 * t3364 * t3085 + 0.2e1 * t2248 * t1600 + t1971 * t1517 + t2949 + 0.2e1 * t159 * t2842 - t3370 * t1436 + 0.4e1 * t3359 * t2853 + 0.4e1 * t1168 * t133 * t995 * t1219 * t2915 - t1081 * t3069 - 0.4e1 * t3195 * t3197 + t2452 + 0.2e1 * t3082 * t1795 - t2719 * t96 - t2589 * t96 + 0.2e1 * t3082 * t1768 - t1444 * t1993 + 0.4e1 * t3367 * t3261 + 0.4e1 * t1922 * t1768 + 0.2e1 * t1075 * t1749 - 0.4e1 * t3071 * t3073 + t2316 + t2180 * t8 - t1851 * t2428 + t2766 + t2825 + t2456 * t87 - t1154 * t1687 - t1154 * t1691 - 0.2e1 * t2491 * t1795 + 0.2e1 * t1696 * t1698 - 0.4e1 * t3533 * t228 + t2385 + t2580 + 0.2e1 * t2458 * t1897 - 0.2e1 * t211 * r_wheelMntRL_Z * t2047 - 0.4e1 * t1550 * t1755 * zFR_zs + 0.2e1 * t1028 * phi_zs1dot * t2347 + r_airRear_Y * t5 * t389 + 0.2e1 * t2832 * psi_zs1dot * t2834 - t18 * t225 * r_wheelMntFL_Z + r_airFront_Y * t5 * t341 - 0.4e1 * t1464 * t1755 * r_wheelMntFL_Z - t31 * t225 * r_wheelMntFR_Z - t31 * t225 * zFR_zs + I_body_zz * phi_zs1dot * t228 - 0.2e1 * t159 * t22 * t1772 * r_wheelMntFL_Y + t22 * r_airRear_X * t389 * t13 - 0.2e1 * t123 * t22 * t1772 * r_wheelMntFR_Y - 0.4e1 * t2400 * t1002 * t5 * theta_zs1dot + t2177 + t3747 + t2796 - 0.2e1 * t1702 * t3659 - 0.2e1 * t2679 * t1795 - t2223 * t96 - t2180 * t14 - 0.2e1 * t1103 * t1861 + 0.2e1 * t2962 * t2963 - t3370 * t1517 - 0.2e1 * t1626 * t1749 - 0.2e1 * t2190 * t1795 + t1639 * t1998 - t1685 * n_gndRL_Y - r_airFront_Z * t13 * t3418 - 0.2e1 * t1122 * t2789 - t3552 * n_gndRR_Y - 0.2e1 * t2116 * theta_zs1dot * t1139 * t22);
gg(5,1) = t86;
gg(5,2) = t510;
gg(5,3) = t817;
gg(5,4) = t1573;
gg(5,5) = (t3782 + t3795 + t3814 + t3842);
gg(5,6) = t3884;
gg(5,7) = -t3885;
gg(5,8) = -t3886;
gg(5,9) = -t3887;
gg(5,10) = -t3888;
gg(5,11) = t3889;
gg(5,12) = t3890;
gg(5,13) = t3891;
gg(5,14) = t3891;
gg(5,15) = (t5197 + t4431 + t4596 + t4898 + t4991 + t4774 + t4634 + t4731 + t4297 + t5313 + t4684 + t3937 + t4558 + t4382 + t5038 + t4815 + t5071 + t4471 + t4094 + t4000 + t5113 + t4202 + t5157 + t4946 + t4857 + t5232 + t4046 + t4513 + t5263 + t4152 + t4249 + t4339);
gg(6,1) = t118;
gg(6,2) = t537;
gg(6,3) = t842;
gg(6,4) = t1656;
gg(6,5) = t3884;
gg(6,6) = (t5319 + t5320);
gg(6,7) = t18;
gg(6,8) = t31;
gg(6,9) = t45;
gg(6,10) = t25;
gg(6,11) = t1670;
gg(6,12) = t1673;
gg(6,15) = (t6267 + t5507 + t6107 + t5701 + t5672 + t5829 + t5921 + t6058 + t5640 + t6186 + t5478 + t5892 + t5613 + t6137 + t6026 + t5734 + t5975 + t5541 + t6002 + t5800 + t5454 + t5576 + t5946 + t6239 + t6084 + t5356 + t5862 + t5766 + t5388 + t6160 + t6211 + t5422);
gg(7,1) = t122;
gg(7,2) = t540;
gg(7,3) = t843;
gg(7,4) = t1660;
gg(7,5) = -t3885;
gg(7,6) = t18;
gg(7,7) = m_wheel;
gg(7,15) = (t6291 + t6311);
gg(8,1) = t122;
gg(8,2) = t540;
gg(8,3) = t843;
gg(8,4) = t1663;
gg(8,5) = -t3886;
gg(8,6) = t31;
gg(8,8) = m_wheel;
gg(8,15) = (t6328 + t6347);
gg(9,1) = t122;
gg(9,2) = t540;
gg(9,3) = t843;
gg(9,4) = t1665;
gg(9,5) = -t3887;
gg(9,6) = t45;
gg(9,9) = m_wheel;
gg(9,15) = (t6365 + t6381);
gg(10,1) = t122;
gg(10,2) = t540;
gg(10,3) = t843;
gg(10,4) = t1667;
gg(10,5) = -t3888;
gg(10,6) = t25;
gg(10,10) = m_wheel;
gg(10,15) = (t6396 + t6416);
gg(11,4) = t1672;
gg(11,5) = t3889;
gg(11,6) = t1670;
gg(11,11) = I_wheel_yy;
gg(11,15) = (-t3745 * t13 * t1925 * n_gndFL_Y - 0.2e1 * t4097 * t6492 + 0.2e1 * t4049 * t2963 - t6421 * t19 * n_gndFL_X - t6421 * t87 * n_gndFL_Y - t6504 * t987 * t4 * t13 * n_gndFL_X - 0.2e1 * t4103 * t2963 + t4069 * t4841 + 0.4e1 * t4097 * t6442 - 0.2e1 * t4107 * t4841 + t6472 - t5448 * t6484 - t5346 * t1917 + t6595 - 0.2e1 * t3932 * t6435 + 0.2e1 * t4510 * t4841 - 0.4e1 * t4407 * t6442 + 0.2e1 * t5770 * t1508 * t1928 + t6528 - 0.2e1 * t5390 * t187 * t1917 + t985 * t164 * t988 + t5759 * t6489 + 0.2e1 * t4101 * t6445 - 0.2e1 * t2381 * t4091 * t6478 + 0.2e1 * t3614 * t6425 + 0.2e1 * t4407 * t6492 + 0.2e1 * t1986 * t5336 - 0.2e1 * t5520 * t6429 + t3857 * t5336 + t6568 + t6616 - t6498 * t6526 + t5105 * t6484 + t5326 * t4268 - 0.2e1 * t5704 * t4268);
gg(12,4) = t1677;
gg(12,5) = t3890;
gg(12,6) = t1673;
gg(12,12) = I_wheel_yy;
gg(12,15) = (-t1712 * t13 * t1697 * n_gndFR_Y - t5448 * t6672 - 0.2e1 * t3109 * t5336 + t3938 * t6648 - 0.2e1 * t5326 * t1004 * t997 * t1039 - t1710 * t1219 * n_gndFR_X + t1712 * t1219 * n_gndFR_Y + 0.4e1 * t3109 * t6456 + t6726 + t6677 * t995 * t12 * t13 * n_gndFR_Y + 0.2e1 * t1036 * t2326 * t1039 - t6653 * t128 * t5344 - t1673 * t5336 + t5326 * t4537 + t4153 * t6738 + 0.2e1 * t6027 * t4537 - t4967 * t6738 + 0.2e1 * t3993 * t6730 + t6823 + t3938 * t6667 + 0.2e1 * t6142 * t6710 - t3945 * t6667 + t6624 * t6626 - t3945 * t6648 + 0.2e1 * t1767 * t6743 - 0.2e1 * t4277 * t1698 + t4069 * t5044 - 0.2e1 * t2557 * t6587 + t5706 * t6635 - t6637 * t6638 - t5346 * t4537 + t6670 + t6772 - t6694 * t5336 + t6794);
gg(13,4) = t1678;
gg(13,5) = t3891;
gg(13,13) = I_wheel_yy;
gg(13,15) = (t6850 + t6867 + t6889 + t6920);
gg(14,4) = t1678;
gg(14,5) = t3891;
gg(14,14) = I_wheel_yy;
gg(14,15) = (t6933 + t6947 + t6976 + t7000);


M=gg(1:14,1:14);
f=-gg(1:14,15);

% second order lag for steering command (poles -5,-5)
%deltaFL2dot = -10*deltaFL_zs1dot-25*deltaFL_zs+25*delta;
%deltaFR2dot = -10*deltaFR_zs1dot-25*deltaFR_zs+25*delta;

% second order lag for steering command (poles -50,-50)
deltaFL2dot = -100*deltaFL_zs1dot-2500*deltaFL_zs+2500*delta;
deltaFR2dot = -100*deltaFR_zs1dot-2500*deltaFR_zs+2500*delta;

q2dot_temp = M\f;

% Assign outputs
q2dot = [q2dot_temp(1:6);deltaFL2dot;deltaFR2dot;q2dot_temp(7:14)];
stuck = [stuckFL;stuckFR;stuckRL;stuckRR];
% R = R (calculated above)

oldepsFL_zs1dot = epsFL_zs1dot;
oldepsFR_zs1dot = epsFR_zs1dot;
oldepsRL_zs1dot = epsRL_zs1dot;
oldepsRR_zs1dot = epsRR_zs1dot;
